simulink model "model"  (R2014a)
(part 4 of 5)

  _CN_227673096_110000_CN_53366641_110000/RConn3 -- T_53366641_220000;110000;6000_ПС_Канаш_220_110_6_кВ/RConn3 -- ВЛ_110_кВ_Канаш_Дружба_CN_53366641_110000_CN_207740804_110000/LConn3 -- ВЛ_110_кВ_Канаш_Дружба_CN_53366641_110000_CN_279846262_110000/LConn3 -- L_53366641/LConn3 -- bus24/LConn1 -- _CN_243154612_110000_CN_53366641_110000/LConn3 -- _CN_262366242_110000_CN_53366641_110000/LConn3 -- _CN_226054226_110000_CN_53366641_110000/LConn3 -- _CN_244847744_110000_CN_53366641_110000/LConn3
  _CN_198002186_110000_CN_197887411_110000/LConn1 -- T_198002186_110000;10000_ПС_110_10_кВ_Бройлерная/LConn1 -- _CN_198002186_110000_CN_311468947_110000/LConn1 -- _CN_198002186_110000_CN_234246987_110000/LConn1 -- _CN_198002186_110000_CN_281834842_110000/LConn1
  _CN_198002186_110000_CN_197887411_110000/LConn2 -- T_198002186_110000;10000_ПС_110_10_кВ_Бройлерная/LConn2 -- _CN_198002186_110000_CN_311468947_110000/LConn2 -- _CN_198002186_110000_CN_234246987_110000/LConn2 -- _CN_198002186_110000_CN_281834842_110000/LConn2
  _CN_198002186_110000_CN_197887411_110000/LConn3 -- T_198002186_110000;10000_ПС_110_10_кВ_Бройлерная/LConn3 -- _CN_198002186_110000_CN_311468947_110000/LConn3 -- _CN_198002186_110000_CN_234246987_110000/LConn3 -- _CN_198002186_110000_CN_281834842_110000/LConn3 -- bus25/LConn1
  _CN_198002186_110000_CN_197887411_110000/RConn1 -- T_197887411_110000;35000;10000_ПС_110_35_10_кВ_Атлашево/LConn1 -- _CN_313773134_110000_CN_197887411_110000/LConn1
  _CN_198002186_110000_CN_197887411_110000/RConn2 -- T_197887411_110000;35000;10000_ПС_110_35_10_кВ_Атлашево/LConn2 -- _CN_313773134_110000_CN_197887411_110000/LConn2
  _CN_198002186_110000_CN_197887411_110000/RConn3 -- T_197887411_110000;35000;10000_ПС_110_35_10_кВ_Атлашево/LConn3 -- _CN_313773134_110000_CN_197887411_110000/LConn3 -- bus26/LConn1
  _CN_198002186_110000_CN_311468947_110000/RConn1 -- T_311468947__ОРУ_ТЭЦ_3/LConn1 -- _CN_313773131_110000_CN_311468947_110000/LConn1 -- _CN_313773134_110000_CN_311468947_110000/LConn1
  _CN_198002186_110000_CN_311468947_110000/RConn2 -- T_311468947__ОРУ_ТЭЦ_3/LConn2 -- _CN_313773131_110000_CN_311468947_110000/LConn2 -- _CN_313773134_110000_CN_311468947_110000/LConn2
  _CN_198002186_110000_CN_311468947_110000/RConn3 -- T_311468947__ОРУ_ТЭЦ_3/LConn3 -- _CN_313773131_110000_CN_311468947_110000/LConn3 -- bus27/LConn1 -- _CN_313773134_110000_CN_311468947_110000/LConn3
  T_234246987_110000;10000_ПС_110_10_кВ_Луч/LConn1 -- _CN_198002186_110000_CN_234246987_110000/RConn1
  T_234246987_110000;10000_ПС_110_10_кВ_Луч/LConn2 -- _CN_198002186_110000_CN_234246987_110000/RConn2
  _CN_198002186_110000_CN_234246987_110000/RConn3 -- T_234246987_110000;10000_ПС_110_10_кВ_Луч/LConn3 -- bus28/LConn1
  _CN_198002186_110000_CN_281834842_110000/RConn1 -- T_281834842_110000;35000;10000_ПС_110_35_10_кВ_Катраси/LConn1 -- ВЛ_110_кВ_Южная_Катраси_CN_281834842_110000_CN_243075861_110000/LConn1 -- _CN_281834842_110000_CN_280247969_110000/RConn1 -- ВЛ_110_кВ_Катраси_Сундырь_с_отпайкой_Россия_CN_281834842_110000_CN_292328535_110000/LConn1 -- ВЛ_110_кВ_Катраси_Сундырь_с_отпайкой_Россия_CN_281834842_110000_CN_292068563_110000/LConn1 -- ВЛ_110_кВ_Катраси_Сундырь_с_отпайкой_Россия_CN_281834842_110000_CN_280247964_110000/LConn1 -- _CN_310752804_110000_CN_281834842_110000/LConn1 -- _CN_281834842_110000_CN_242972920_110000/LConn1 -- _CN_281834842_110000_CN_242973735_110000/LConn1
  _CN_198002186_110000_CN_281834842_110000/RConn2 -- T_281834842_110000;35000;10000_ПС_110_35_10_кВ_Катраси/LConn2 -- ВЛ_110_кВ_Южная_Катраси_CN_281834842_110000_CN_243075861_110000/LConn2 -- _CN_281834842_110000_CN_280247969_110000/RConn2 -- ВЛ_110_кВ_Катраси_Сундырь_с_отпайкой_Россия_CN_281834842_110000_CN_292328535_110000/LConn2 -- ВЛ_110_кВ_Катраси_Сундырь_с_отпайкой_Россия_CN_281834842_110000_CN_292068563_110000/LConn2 -- ВЛ_110_кВ_Катраси_Сундырь_с_отпайкой_Россия_CN_281834842_110000_CN_280247964_110000/LConn2 -- _CN_310752804_110000_CN_281834842_110000/LConn2 -- _CN_281834842_110000_CN_242972920_110000/LConn2 -- _CN_281834842_110000_CN_242973735_110000/LConn2
  _CN_198002186_110000_CN_281834842_110000/RConn3 -- T_281834842_110000;35000;10000_ПС_110_35_10_кВ_Катраси/LConn3 -- ВЛ_110_кВ_Южная_Катраси_CN_281834842_110000_CN_243075861_110000/LConn3 -- bus29/LConn1 -- _CN_281834842_110000_CN_280247969_110000/RConn3 -- ВЛ_110_кВ_Катраси_Сундырь_с_отпайкой_Россия_CN_281834842_110000_CN_292328535_110000/LConn3 -- ВЛ_110_кВ_Катраси_Сундырь_с_отпайкой_Россия_CN_281834842_110000_CN_292068563_110000/LConn3 -- ВЛ_110_кВ_Катраси_Сундырь_с_отпайкой_Россия_CN_281834842_110000_CN_280247964_110000/LConn3 -- _CN_310752804_110000_CN_281834842_110000/LConn3 -- _CN_281834842_110000_CN_242972920_110000/LConn3 -- _CN_281834842_110000_CN_242973735_110000/LConn3
  T_180390411__ПС_Бугульма/LConn1 -- ВЛ_Бугульма___Карабаш_II_110кВ_CN_180390411_110000_CN_238549570_110000/LConn1
  T_180390411__ПС_Бугульма/LConn2 -- ВЛ_Бугульма___Карабаш_II_110кВ_CN_180390411_110000_CN_238549570_110000/LConn2
  ВЛ_Бугульма___Карабаш_II_110кВ_CN_180390411_110000_CN_238549570_110000/LConn3 -- T_180390411__ПС_Бугульма/LConn3 -- bus30/LConn1
  T_238549570__ПС_Алкино/LConn1 -- ВЛ_Бугульма___Карабаш_II_110кВ_CN_180390411_110000_CN_238549570_110000/RConn1
  T_238549570__ПС_Алкино/LConn2 -- ВЛ_Бугульма___Карабаш_II_110кВ_CN_180390411_110000_CN_238549570_110000/RConn2
  ВЛ_Бугульма___Карабаш_II_110кВ_CN_180390411_110000_CN_238549570_110000/RConn3 -- T_238549570__ПС_Алкино/LConn3 -- bus31/LConn1
  T_82459148_110000_ОРУ_110_кВ/LConn1 -- _CN_82459148_110000_CN_273327356_110000/LConn1
  T_82459148_110000_ОРУ_110_кВ/LConn2 -- _CN_82459148_110000_CN_273327356_110000/LConn2
  _CN_82459148_110000_CN_273327356_110000/LConn3 -- T_82459148_110000_ОРУ_110_кВ/LConn3 -- bus32/LConn1
  _CN_82459148_110000_CN_273327356_110000/RConn1 -- G_273327356_Воткинская_ГЭС/RConn1 -- _CN_82458858_220000_CN_273327356_110000/LConn1 -- _CN_82459105_500000_CN_273327356_110000/LConn1
  _CN_82459148_110000_CN_273327356_110000/RConn2 -- G_273327356_Воткинская_ГЭС/RConn2 -- _CN_82458858_220000_CN_273327356_110000/LConn2 -- _CN_82459105_500000_CN_273327356_110000/LConn2
  _CN_82459148_110000_CN_273327356_110000/RConn3 -- G_273327356_Воткинская_ГЭС/RConn3 -- _CN_82458858_220000_CN_273327356_110000/LConn3 -- _CN_82459105_500000_CN_273327356_110000/LConn3 -- bus33/LConn1
  _CN_104554513_110000_CN_320965592_110000/LConn1 -- T_104554513__/LConn1 -- _CN_104554513_110000_CN_93482528_110000/LConn1 -- _CN_104554513_110000_CN_67498838_110000/RConn1
  _CN_104554513_110000_CN_320965592_110000/LConn2 -- T_104554513__/LConn2 -- _CN_104554513_110000_CN_93482528_110000/LConn2 -- _CN_104554513_110000_CN_67498838_110000/RConn2
  _CN_104554513_110000_CN_320965592_110000/LConn3 -- T_104554513__/LConn3 -- _CN_104554513_110000_CN_93482528_110000/LConn3 -- _CN_104554513_110000_CN_67498838_110000/RConn3 -- bus34/LConn1
  _CN_104554513_110000_CN_320965592_110000/RConn1 -- T_320965592__/LConn1 -- _CN_67498838_110000_CN_320965592_110000/RConn1
  _CN_104554513_110000_CN_320965592_110000/RConn2 -- T_320965592__/LConn2 -- _CN_67498838_110000_CN_320965592_110000/RConn2
  _CN_104554513_110000_CN_320965592_110000/RConn3 -- T_320965592__/LConn3 -- _CN_67498838_110000_CN_320965592_110000/RConn3 -- bus35/LConn1
  T_93482528__/LConn1 -- _CN_104554513_110000_CN_93482528_110000/RConn1
  T_93482528__/LConn2 -- _CN_104554513_110000_CN_93482528_110000/RConn2
  _CN_104554513_110000_CN_93482528_110000/RConn3 -- T_93482528__/LConn3 -- bus36/LConn1
  T_158349331__/LConn1 -- _CN_158349331_110000_CN_109525418_110000/LConn1
  T_158349331__/LConn2 -- _CN_158349331_110000_CN_109525418_110000/LConn2
  _CN_158349331_110000_CN_109525418_110000/LConn3 -- T_158349331__/LConn3 -- bus37/LConn1
  _CN_158349331_110000_CN_109525418_110000/RConn1 -- T_109525418_220000_Подстанция_220_кВ_Титан/LConn1 -- _CN_172819864_110000_CN_109525418_110000/LConn1 -- _CN_193928464_110000_CN_109525418_110000/LConn1 -- _CN_97060032_110000_CN_109525418_110000/LConn1 -- _CN_97060037_110000_CN_109525418_110000/LConn1
  _CN_158349331_110000_CN_109525418_110000/RConn2 -- T_109525418_220000_Подстанция_220_кВ_Титан/LConn2 -- _CN_172819864_110000_CN_109525418_110000/LConn2 -- _CN_193928464_110000_CN_109525418_110000/LConn2 -- _CN_97060032_110000_CN_109525418_110000/LConn2 -- _CN_97060037_110000_CN_109525418_110000/LConn2
  _CN_158349331_110000_CN_109525418_110000/RConn3 -- T_109525418_220000_Подстанция_220_кВ_Титан/LConn3 -- _CN_172819864_110000_CN_109525418_110000/LConn3 -- bus38/LConn1 -- _CN_193928464_110000_CN_109525418_110000/LConn3 -- _CN_97060032_110000_CN_109525418_110000/LConn3 -- _CN_97060037_110000_CN_109525418_110000/LConn3
  T_330052123_110000_ПС_110_6_кВ_Прудовая/LConn1 -- _CN_330052123_110000_CN_116695201_110000/LConn1
  T_330052123_110000_ПС_110_6_кВ_Прудовая/LConn2 -- _CN_330052123_110000_CN_116695201_110000/LConn2
  _CN_330052123_110000_CN_116695201_110000/LConn3 -- T_330052123_110000_ПС_110_6_кВ_Прудовая/LConn3 -- bus39/LConn1
  _CN_330052123_110000_CN_116695201_110000/RConn1 -- T_116695201_110000_ПС_110_35_6_Воткинск/LConn1 -- _CN_330006647_110000_CN_116695201_110000/LConn1 -- _CN_172508720_110000_CN_116695201_110000/LConn1
  _CN_330052123_110000_CN_116695201_110000/RConn2 -- T_116695201_110000_ПС_110_35_6_Воткинск/LConn2 -- _CN_330006647_110000_CN_116695201_110000/LConn2 -- _CN_172508720_110000_CN_116695201_110000/LConn2
  _CN_330052123_110000_CN_116695201_110000/RConn3 -- T_116695201_110000_ПС_110_35_6_Воткинск/LConn3 -- _CN_330006647_110000_CN_116695201_110000/LConn3 -- bus40/LConn1 -- _CN_172508720_110000_CN_116695201_110000/LConn3
  _CN_262366242_110000_CN_208425687_110000/LConn1 -- T_262366242_110000;35000;10000_ПС_110_35_10_кВ_Батырево/LConn1 -- _CN_262366242_110000_CN_53366641_110000/RConn1 -- _CN_262366242_110000_CN_243068515_110000/LConn1 -- _CN_262366242_110000_CN_279919300_110000/RConn1 -- _CN_262366242_110000_CN_262366241_110000/LConn1
  _CN_262366242_110000_CN_208425687_110000/LConn2 -- T_262366242_110000;35000;10000_ПС_110_35_10_кВ_Батырево/LConn2 -- _CN_262366242_110000_CN_53366641_110000/RConn2 -- _CN_262366242_110000_CN_243068515_110000/LConn2 -- _CN_262366242_110000_CN_279919300_110000/RConn2 -- _CN_262366242_110000_CN_262366241_110000/LConn2
  _CN_262366242_110000_CN_208425687_110000/LConn3 -- T_262366242_110000;35000;10000_ПС_110_35_10_кВ_Батырево/LConn3 -- _CN_262366242_110000_CN_53366641_110000/RConn3 -- _CN_262366242_110000_CN_243068515_110000/LConn3 -- _CN_262366242_110000_CN_279919300_110000/RConn3 -- _CN_262366242_110000_CN_262366241_110000/LConn3 -- bus41/LConn1
  T_208425687_110000;35000;10000_ПС_110_35_10_кВ_Комсомольская/LConn1 -- _CN_262366242_110000_CN_208425687_110000/RConn1
  T_208425687_110000;35000;10000_ПС_110_35_10_кВ_Комсомольская/LConn2 -- _CN_262366242_110000_CN_208425687_110000/RConn2
  _CN_262366242_110000_CN_208425687_110000/RConn3 -- T_208425687_110000;35000;10000_ПС_110_35_10_кВ_Комсомольская/LConn3 -- bus42/LConn1
  T_243068515_110000;10000_ПС_110_10_кВ_Маяк/LConn1 -- _CN_262366242_110000_CN_243068515_110000/RConn1
  T_243068515_110000;10000_ПС_110_10_кВ_Маяк/LConn2 -- _CN_262366242_110000_CN_243068515_110000/RConn2
  _CN_262366242_110000_CN_243068515_110000/RConn3 -- T_243068515_110000;10000_ПС_110_10_кВ_Маяк/LConn3 -- bus43/LConn1
  _CN_262366242_110000_CN_262366241_110000/RConn1 -- T_262366241_110000;10000_ПС_110_10_кВ_Сугуты/LConn1 -- _CN_194431022_110000_CN_262366241_110000/LConn1
  _CN_262366242_110000_CN_262366241_110000/RConn2 -- T_262366241_110000;10000_ПС_110_10_кВ_Сугуты/LConn2 -- _CN_194431022_110000_CN_262366241_110000/LConn2
  _CN_262366242_110000_CN_262366241_110000/RConn3 -- T_262366241_110000;10000_ПС_110_10_кВ_Сугуты/LConn3 -- _CN_194431022_110000_CN_262366241_110000/LConn3 -- bus44/LConn1
  _CN_310752804_110000_CN_281834842_110000/RConn1 -- T_310752804_110000;35000;10000_ПС_«Чапаевская»_110_35_10_кВ/LConn1 -- _CN_310752804_110000_CN_243075861_110000/LConn1
  _CN_310752804_110000_CN_281834842_110000/RConn2 -- T_310752804_110000;35000;10000_ПС_«Чапаевская»_110_35_10_кВ/LConn2 -- _CN_310752804_110000_CN_243075861_110000/LConn2
  _CN_310752804_110000_CN_281834842_110000/RConn3 -- T_310752804_110000;35000;10000_ПС_«Чапаевская»_110_35_10_кВ/LConn3 -- _CN_310752804_110000_CN_243075861_110000/LConn3 -- bus45/LConn1
  _CN_310752804_110000_CN_243075861_110000/RConn1 -- T_243075861_110000;6000_ПС_110_6_кВ_Южная/LConn1 -- ВЛ_110_кВ_Южная_Катраси_CN_281834842_110000_CN_243075861_110000/RConn1
  _CN_310752804_110000_CN_243075861_110000/RConn2 -- T_243075861_110000;6000_ПС_110_6_кВ_Южная/LConn2 -- ВЛ_110_кВ_Южная_Катраси_CN_281834842_110000_CN_243075861_110000/RConn2
  _CN_310752804_110000_CN_243075861_110000/RConn3 -- T_243075861_110000;6000_ПС_110_6_кВ_Южная/LConn3 -- ВЛ_110_кВ_Южная_Катраси_CN_281834842_110000_CN_243075861_110000/RConn3 -- bus46/LConn1
  _CN_97124903_110000_CN_145399632_110000/LConn1 -- T_97124903__/LConn1 -- _CN_97124903_110000_CN_97124768_110000/LConn1
  _CN_97124903_110000_CN_145399632_110000/LConn2 -- T_97124903__/LConn2 -- _CN_97124903_110000_CN_97124768_110000/LConn2
  _CN_97124903_110000_CN_145399632_110000/LConn3 -- T_97124903__/LConn3 -- _CN_97124903_110000_CN_97124768_110000/LConn3 -- bus47/LConn1
  T_145399632__/LConn1 -- _CN_97124903_110000_CN_145399632_110000/RConn1
  T_145399632__/LConn2 -- _CN_97124903_110000_CN_145399632_110000/RConn2
  _CN_97124903_110000_CN_145399632_110000/RConn3 -- T_145399632__/LConn3 -- bus48/LConn1
  T_97124768__/LConn1 -- _CN_97124903_110000_CN_97124768_110000/RConn1
  T_97124768__/LConn2 -- _CN_97124903_110000_CN_97124768_110000/RConn2
  _CN_97124903_110000_CN_97124768_110000/RConn3 -- T_97124768__/LConn3 -- bus49/LConn1
  _CN_279978588_110000_CN_279978582_110000/LConn1 -- T_279978588_110000;10000_ПС_110_10_кВ_Алгаши/LConn1 -- _CN_279978588_110000_CN_279978583_110000/LConn1 -- _CN_279978588_110000_CN_207204995_110000/LConn1
  _CN_279978588_110000_CN_279978582_110000/LConn2 -- T_279978588_110000;10000_ПС_110_10_кВ_Алгаши/LConn2 -- _CN_279978588_110000_CN_279978583_110000/LConn2 -- _CN_279978588_110000_CN_207204995_110000/LConn2
  _CN_279978588_110000_CN_279978582_110000/LConn3 -- T_279978588_110000;10000_ПС_110_10_кВ_Алгаши/LConn3 -- _CN_279978588_110000_CN_279978583_110000/LConn3 -- _CN_279978588_110000_CN_207204995_110000/LConn3 -- bus50/LConn1
  _CN_279978588_110000_CN_279978582_110000/RConn1 -- T_279978582_110000;35000;10000_ПС_110_35_10_кВ_Порецкая/LConn1 -- _CN_279978581_110000_CN_279978582_110000/LConn1
  _CN_279978588_110000_CN_279978582_110000/RConn2 -- T_279978582_110000;35000;10000_ПС_110_35_10_кВ_Порецкая/LConn2 -- _CN_279978581_110000_CN_279978582_110000/LConn2
  _CN_279978588_110000_CN_279978582_110000/RConn3 -- T_279978582_110000;35000;10000_ПС_110_35_10_кВ_Порецкая/LConn3 -- _CN_279978581_110000_CN_279978582_110000/LConn3 -- bus51/LConn1
  T_279978583_110000;10000_ПС_110_10_кВ_Кожевенная/LConn1 -- _CN_279978588_110000_CN_279978583_110000/RConn1
  T_279978583_110000;10000_ПС_110_10_кВ_Кожевенная/LConn2 -- _CN_279978588_110000_CN_279978583_110000/RConn2
  _CN_279978588_110000_CN_279978583_110000/RConn3 -- T_279978583_110000;10000_ПС_110_10_кВ_Кожевенная/LConn3 -- bus52/LConn1
  _CN_279978588_110000_CN_207204995_110000/RConn1 -- T_207204995_220000;110000;6000_ПС_Венец_220_110_6_кВ/RConn1 -- _CN_244847744_110000_CN_207204995_110000/LConn1 -- _CN_207204995_110000_CN_207206840_110000/LConn1 -- L_207204995/LConn1
  _CN_279978588_110000_CN_207204995_110000/RConn2 -- T_207204995_220000;110000;6000_ПС_Венец_220_110_6_кВ/RConn2 -- _CN_244847744_110000_CN_207204995_110000/LConn2 -- _CN_207204995_110000_CN_207206840_110000/LConn2 -- L_207204995/LConn2
  _CN_279978588_110000_CN_207204995_110000/RConn3 -- T_207204995_220000;110000;6000_ПС_Венец_220_110_6_кВ/RConn3 -- _CN_244847744_110000_CN_207204995_110000/LConn3 -- _CN_207204995_110000_CN_207206840_110000/LConn3 -- L_207204995/LConn3 -- bus53/LConn1
  _CN_250911823_110000_CN_351596015_110000/LConn1 -- T_250911823__ПС_Б_Матаки/LConn1 -- _CN_250911823_110000_CN_183273018_110000/LConn1
  _CN_250911823_110000_CN_351596015_110000/LConn2 -- T_250911823__ПС_Б_Матаки/LConn2 -- _CN_250911823_110000_CN_183273018_110000/LConn2
  _CN_250911823_110000_CN_351596015_110000/LConn3 -- T_250911823__ПС_Б_Матаки/LConn3 -- _CN_250911823_110000_CN_183273018_110000/LConn3 -- bus54/LConn1
  T_351596015__ПС_Ромодан/LConn1 -- _CN_250911823_110000_CN_351596015_110000/RConn1
  T_351596015__ПС_Ромодан/LConn2 -- _CN_250911823_110000_CN_351596015_110000/RConn2
  _CN_250911823_110000_CN_351596015_110000/RConn3 -- T_351596015__ПС_Ромодан/LConn3 -- bus55/LConn1
  T_183273018__ПС_Салманы/LConn1 -- _CN_250911823_110000_CN_183273018_110000/RConn1
  T_183273018__ПС_Салманы/LConn2 -- _CN_250911823_110000_CN_183273018_110000/RConn2
  _CN_250911823_110000_CN_183273018_110000/RConn3 -- T_183273018__ПС_Салманы/LConn3 -- bus56/LConn1
  _CN_194431022_110000_CN_262366241_110000/RConn1 -- T_194431022_110000;35000;10000_ПС_110_35_10_кВ_Яльчики/LConn1 -- _CN_194431022_110000_CN_279778884_110000/LConn1
  _CN_194431022_110000_CN_262366241_110000/RConn2 -- T_194431022_110000;35000;10000_ПС_110_35_10_кВ_Яльчики/LConn2 -- _CN_194431022_110000_CN_279778884_110000/LConn2
  _CN_194431022_110000_CN_262366241_110000/RConn3 -- T_194431022_110000;35000;10000_ПС_110_35_10_кВ_Яльчики/LConn3 -- _CN_194431022_110000_CN_279778884_110000/LConn3 -- bus57/LConn1
  T_279778884_110000;10000_ПС_110_10_кВ_Слава/LConn1 -- _CN_194431022_110000_CN_279778884_110000/RConn1
  T_279778884_110000;10000_ПС_110_10_кВ_Слава/LConn2 -- _CN_194431022_110000_CN_279778884_110000/RConn2
  _CN_194431022_110000_CN_279778884_110000/RConn3 -- T_279778884_110000;10000_ПС_110_10_кВ_Слава/LConn3 -- bus58/LConn1
  T_172508720_110000_ПС_110_10_Успенка/LConn1 -- _CN_172508720_110000_CN_116695201_110000/RConn1
  T_172508720_110000_ПС_110_10_Успенка/LConn2 -- _CN_172508720_110000_CN_116695201_110000/RConn2
  _CN_172508720_110000_CN_116695201_110000/RConn3 -- T_172508720_110000_ПС_110_10_Успенка/LConn3 -- bus59/LConn1
  _CN_157080628_110000_CN_192432407_110000/LConn1 -- T_157080628__/LConn1 -- _CN_157080628_110000_CN_192432406_110000/LConn1 -- _CN_157080628_110000_CN_192426717_110000/LConn1
  _CN_157080628_110000_CN_192432407_110000/LConn2 -- T_157080628__/LConn2 -- _CN_157080628_110000_CN_192432406_110000/LConn2 -- _CN_157080628_110000_CN_192426717_110000/LConn2
  _CN_157080628_110000_CN_192432407_110000/LConn3 -- T_157080628__/LConn3 -- _CN_157080628_110000_CN_192432406_110000/LConn3 -- _CN_157080628_110000_CN_192426717_110000/LConn3 -- bus60/LConn1
  T_192432407__/LConn1 -- _CN_157080628_110000_CN_192432407_110000/RConn1
  T_192432407__/LConn2 -- _CN_157080628_110000_CN_192432407_110000/RConn2
  _CN_157080628_110000_CN_192432407_110000/RConn3 -- T_192432407__/LConn3 -- bus61/LConn1
  T_192432406__/LConn1 -- _CN_157080628_110000_CN_192432406_110000/RConn1
  T_192432406__/LConn2 -- _CN_157080628_110000_CN_192432406_110000/RConn2
  _CN_157080628_110000_CN_192432406_110000/RConn3 -- T_192432406__/LConn3 -- bus62/LConn1
  T_192426717_110000_ПС_Люзень/LConn1 -- _CN_157080628_110000_CN_192426717_110000/RConn1
  T_192426717_110000_ПС_Люзень/LConn2 -- _CN_157080628_110000_CN_192426717_110000/RConn2
  _CN_157080628_110000_CN_192426717_110000/RConn3 -- T_192426717_110000_ПС_Люзень/LConn3 -- bus63/LConn1
  T_236703070__ПС_Дубъязы/LConn1 -- ВЛ_Дубъязы___Алат_110кВ_CN_236703070_110000_CN_180786877_110000/LConn1
  T_236703070__ПС_Дубъязы/LConn2 -- ВЛ_Дубъязы___Алат_110кВ_CN_236703070_110000_CN_180786877_110000/LConn2
  ВЛ_Дубъязы___Алат_110кВ_CN_236703070_110000_CN_180786877_110000/LConn3 -- T_236703070__ПС_Дубъязы/LConn3 -- bus64/LConn1
  T_180786877__ПС_Алат/LConn1 -- ВЛ_Дубъязы___Алат_110кВ_CN_236703070_110000_CN_180786877_110000/RConn1
  T_180786877__ПС_Алат/LConn2 -- ВЛ_Дубъязы___Алат_110кВ_CN_236703070_110000_CN_180786877_110000/RConn2
  ВЛ_Дубъязы___Алат_110кВ_CN_236703070_110000_CN_180786877_110000/RConn3 -- T_180786877__ПС_Алат/LConn3 -- bus65/LConn1
  T_291372086_110000_пс_Села_110_10кВ/LConn1 -- _CN_291372086_110000_CN_291372085_110000/LConn1
  T_291372086_110000_пс_Села_110_10кВ/LConn2 -- _CN_291372086_110000_CN_291372085_110000/LConn2
  _CN_291372086_110000_CN_291372085_110000/LConn3 -- T_291372086_110000_пс_Села_110_10кВ/LConn3 -- bus66/LConn1
  T_291372085_110000_пс_Кутамыш/LConn1 -- _CN_291372086_110000_CN_291372085_110000/RConn1
  T_291372085_110000_пс_Кутамыш/LConn2 -- _CN_291372086_110000_CN_291372085_110000/RConn2
  _CN_291372086_110000_CN_291372085_110000/RConn3 -- T_291372085_110000_пс_Кутамыш/LConn3 -- bus67/LConn1
  _CN_277905350_110000_CN_277905349_110000/LConn1 -- T_277905350_220000;110000_Сергач/RConn1 -- L_277905350/LConn1
  _CN_277905350_110000_CN_277905349_110000/LConn2 -- T_277905350_220000;110000_Сергач/RConn2 -- L_277905350/LConn2
  _CN_277905350_110000_CN_277905349_110000/LConn3 -- T_277905350_220000;110000_Сергач/RConn3 -- L_277905350/LConn3 -- bus68/LConn1
  T_277905349_110000;10000_Андреевка/LConn1 -- _CN_277905350_110000_CN_277905349_110000/RConn1
  T_277905349_110000;10000_Андреевка/LConn2 -- _CN_277905350_110000_CN_277905349_110000/RConn2
  _CN_277905350_110000_CN_277905349_110000/RConn3 -- T_277905349_110000;10000_Андреевка/LConn3 -- bus69/LConn1
  _CN_281834842_110000_CN_242972920_110000/RConn1 -- T_242972920_110000;10000_ПС_110_10_кВ_Заволжская/LConn1 -- _CN_279258960_110000_CN_242972920_110000/LConn1
  _CN_281834842_110000_CN_242972920_110000/RConn2 -- T_242972920_110000;10000_ПС_110_10_кВ_Заволжская/LConn2 -- _CN_279258960_110000_CN_242972920_110000/LConn2
  _CN_281834842_110000_CN_242972920_110000/RConn3 -- T_242972920_110000;10000_ПС_110_10_кВ_Заволжская/LConn3 -- _CN_279258960_110000_CN_242972920_110000/LConn3 -- bus70/LConn1
  T_242973735_110000;10000_ПС_110_10_кВ_Яндоба/LConn1 -- _CN_281834842_110000_CN_242973735_110000/RConn1
  T_242973735_110000;10000_ПС_110_10_кВ_Яндоба/LConn2 -- _CN_281834842_110000_CN_242973735_110000/RConn2
  _CN_281834842_110000_CN_242973735_110000/RConn3 -- T_242973735_110000;10000_ПС_110_10_кВ_Яндоба/LConn3 -- bus71/LConn1
  T_292328535_110000;10000_ПС_110_10_кВ_Виловатово/LConn1 -- ВЛ_110_кВ_Катраси_Сундырь_с_отпайкой_Россия_CN_281834842_110000_CN_292328535_110000/RConn1
  T_292328535_110000;10000_ПС_110_10_кВ_Виловатово/LConn2 -- ВЛ_110_кВ_Катраси_Сундырь_с_отпайкой_Россия_CN_281834842_110000_CN_292328535_110000/RConn2
  ВЛ_110_кВ_Катраси_Сундырь_с_отпайкой_Россия_CN_281834842_110000_CN_292328535_110000/RConn3 -- T_292328535_110000;10000_ПС_110_10_кВ_Виловатово/LConn3 -- bus72/LConn1
  T_292068563_110000;35000;10000_ПС_110_35_10_кВ_Еласы/LConn1 -- ВЛ_110_кВ_Катраси_Сундырь_с_отпайкой_Россия_CN_281834842_110000_CN_292068563_110000/RConn1
  T_292068563_110000;35000;10000_ПС_110_35_10_кВ_Еласы/LConn2 -- ВЛ_110_кВ_Катраси_Сундырь_с_отпайкой_Россия_CN_281834842_110000_CN_292068563_110000/RConn2
  ВЛ_110_кВ_Катраси_Сундырь_с_отпайкой_Россия_CN_281834842_110000_CN_292068563_110000/RConn3 -- T_292068563_110000;35000;10000_ПС_110_35_10_кВ_Еласы/LConn3 -- bus73/LConn1
  T_280247964_110000;10000_ПС_110_10_кВ_Сундырь/LConn1 -- ВЛ_110_кВ_Катраси_Сундырь_с_отпайкой_Россия_CN_281834842_110000_CN_280247964_110000/RConn1
  T_280247964_110000;10000_ПС_110_10_кВ_Сундырь/LConn2 -- ВЛ_110_кВ_Катраси_Сундырь_с_отпайкой_Россия_CN_281834842_110000_CN_280247964_110000/RConn2
  ВЛ_110_кВ_Катраси_Сундырь_с_отпайкой_Россия_CN_281834842_110000_CN_280247964_110000/RConn3 -- T_280247964_110000;10000_ПС_110_10_кВ_Сундырь/LConn3 -- bus74/LConn1
  T_226055229_110000;10000_ПС_110_10_кВ_Козловка/LConn1 -- ВЛ_Тюрлема___Козловка_110кВ_CN_226055229_110000_CN_121218185_110000/LConn1
  T_226055229_110000;10000_ПС_110_10_кВ_Козловка/LConn2 -- ВЛ_Тюрлема___Козловка_110кВ_CN_226055229_110000_CN_121218185_110000/LConn2
  ВЛ_Тюрлема___Козловка_110кВ_CN_226055229_110000_CN_121218185_110000/LConn3 -- T_226055229_110000;10000_ПС_110_10_кВ_Козловка/LConn3 -- bus75/LConn1
  ВЛ_Тюрлема___Козловка_110кВ_CN_226055229_110000_CN_121218185_110000/RConn1 -- T_121218185_220000;110000;10000_ПС_220_110_10_кВ_Тюрлема/RConn1 -- _CN_121218185_110000_CN_226055643_110000/LConn1 -- L_121218185/LConn1 -- ВЛ_Свияжск___Тюрлема_110кВ_CN_121218185_110000_CN_191841753_110000/LConn1 -- ВЛ_Нурлаты___Федоровская_110_кВ_CN_120823877_110000_CN_121218185_110000/LConn1 -- _CN_226054226_110000_CN_121218185_110000/LConn1
  ВЛ_Тюрлема___Козловка_110кВ_CN_226055229_110000_CN_121218185_110000/RConn2 -- T_121218185_220000;110000;10000_ПС_220_110_10_кВ_Тюрлема/RConn2 -- _CN_121218185_110000_CN_226055643_110000/LConn2 -- L_121218185/LConn2 -- ВЛ_Свияжск___Тюрлема_110кВ_CN_121218185_110000_CN_191841753_110000/LConn2 -- ВЛ_Нурлаты___Федоровская_110_кВ_CN_120823877_110000_CN_121218185_110000/LConn2 -- _CN_226054226_110000_CN_121218185_110000/LConn2
  ВЛ_Тюрлема___Козловка_110кВ_CN_226055229_110000_CN_121218185_110000/RConn3 -- T_121218185_220000;110000;10000_ПС_220_110_10_кВ_Тюрлема/RConn3 -- _CN_121218185_110000_CN_226055643_110000/LConn3 -- L_121218185/LConn3 -- bus76/LConn1 -- ВЛ_Свияжск___Тюрлема_110кВ_CN_121218185_110000_CN_191841753_110000/LConn3 -- ВЛ_Нурлаты___Федоровская_110_кВ_CN_120823877_110000_CN_121218185_110000/LConn3 -- _CN_226054226_110000_CN_121218185_110000/LConn3
  _CN_115651649_110000_CN_281879368_110000/LConn1 -- T_115651649_110000;10000_ПС_110_10_кВ_Вурманкасы/LConn1 -- _CN_115651649_110000_CN_281834847_110000/LConn1
  _CN_115651649_110000_CN_281879368_110000/LConn2 -- T_115651649_110000;10000_ПС_110_10_кВ_Вурманкасы/LConn2 -- _CN_115651649_110000_CN_281834847_110000/LConn2
  _CN_115651649_110000_CN_281879368_110000/LConn3 -- T_115651649_110000;10000_ПС_110_10_кВ_Вурманкасы/LConn3 -- _CN_115651649_110000_CN_281834847_110000/LConn3 -- bus77/LConn1
  T_281879368_110000;10000_ПС_110_10_кВ_Радуга/LConn1 -- _CN_115651649_110000_CN_281879368_110000/RConn1
  T_281879368_110000;10000_ПС_110_10_кВ_Радуга/LConn2 -- _CN_115651649_110000_CN_281879368_110000/RConn2
  _CN_115651649_110000_CN_281879368_110000/RConn3 -- T_281879368_110000;10000_ПС_110_10_кВ_Радуга/LConn3 -- bus78/LConn1
  T_281834847_110000;35000;10000_ПС_110_35_10_кВ_Кугеси/LConn1 -- _CN_115651649_110000_CN_281834847_110000/RConn1
  T_281834847_110000;35000;10000_ПС_110_35_10_кВ_Кугеси/LConn2 -- _CN_115651649_110000_CN_281834847_110000/RConn2
  _CN_115651649_110000_CN_281834847_110000/RConn3 -- T_281834847_110000;35000;10000_ПС_110_35_10_кВ_Кугеси/LConn3 -- bus79/LConn1
  ВЛ_Нурлаты___Федоровская_110_кВ_CN_120823877_110000_CN_229841888_110000/LConn1 -- T_120823877__ПС_Федоровская/LConn1 -- ВЛ_Нурлаты___Федоровская_110_кВ_CN_120823877_110000_CN_121218185_110000/RConn1 -- ВЛ_Нурлаты___Федоровская_110_кВ_CN_120823877_110000_CN_171977680_110000/LConn1 -- ВЛ_Нурлаты___Федоровская_110_кВ_CN_120823877_110000_CN_176838936_110000/LConn1
  ВЛ_Нурлаты___Федоровская_110_кВ_CN_120823877_110000_CN_229841888_110000/LConn2 -- T_120823877__ПС_Федоровская/LConn2 -- ВЛ_Нурлаты___Федоровская_110_кВ_CN_120823877_110000_CN_121218185_110000/RConn2 -- ВЛ_Нурлаты___Федоровская_110_кВ_CN_120823877_110000_CN_171977680_110000/LConn2 -- ВЛ_Нурлаты___Федоровская_110_кВ_CN_120823877_110000_CN_176838936_110000/LConn2
  ВЛ_Нурлаты___Федоровская_110_кВ_CN_120823877_110000_CN_229841888_110000/LConn3 -- T_120823877__ПС_Федоровская/LConn3 -- ВЛ_Нурлаты___Федоровская_110_кВ_CN_120823877_110000_CN_121218185_110000/RConn3 -- ВЛ_Нурлаты___Федоровская_110_кВ_CN_120823877_110000_CN_171977680_110000/LConn3 -- ВЛ_Нурлаты___Федоровская_110_кВ_CN_120823877_110000_CN_176838936_110000/LConn3 -- bus80/LConn1
  T_229841888__ПС_Нурлаты/LConn1 -- ВЛ_Нурлаты___Федоровская_110_кВ_CN_120823877_110000_CN_229841888_110000/RConn1
  T_229841888__ПС_Нурлаты/LConn2 -- ВЛ_Нурлаты___Федоровская_110_кВ_CN_120823877_110000_CN_229841888_110000/RConn2
  ВЛ_Нурлаты___Федоровская_110_кВ_CN_120823877_110000_CN_229841888_110000/RConn3 -- T_229841888__ПС_Нурлаты/LConn3 -- bus81/LConn1
  ВЛ_Нурлаты___Федоровская_110_кВ_CN_120823877_110000_CN_171977680_110000/RConn1 -- T_171977680__ПС_Апастово/LConn1 -- _CN_113994637_110000_CN_171977680_110000/LConn1
  ВЛ_Нурлаты___Федоровская_110_кВ_CN_120823877_110000_CN_171977680_110000/RConn2 -- T_171977680__ПС_Апастово/LConn2 -- _CN_113994637_110000_CN_171977680_110000/LConn2
  ВЛ_Нурлаты___Федоровская_110_кВ_CN_120823877_110000_CN_171977680_110000/RConn3 -- T_171977680__ПС_Апастово/LConn3 -- _CN_113994637_110000_CN_171977680_110000/LConn3 -- bus82/LConn1
  T_176838936__ПС_Каратун/LConn1 -- ВЛ_Нурлаты___Федоровская_110_кВ_CN_120823877_110000_CN_176838936_110000/RConn1
  T_176838936__ПС_Каратун/LConn2 -- ВЛ_Нурлаты___Федоровская_110_кВ_CN_120823877_110000_CN_176838936_110000/RConn2
  ВЛ_Нурлаты___Федоровская_110_кВ_CN_120823877_110000_CN_176838936_110000/RConn3 -- T_176838936__ПС_Каратун/LConn3 -- bus83/LConn1
  T_94242892__Подстанция_№3/LConn1 -- _CN_94242892_110000_CN_97145033_110000/LConn1
  T_94242892__Подстанция_№3/LConn2 -- _CN_94242892_110000_CN_97145033_110000/LConn2
  _CN_94242892_110000_CN_97145033_110000/LConn3 -- T_94242892__Подстанция_№3/LConn3 -- bus84/LConn1
  _CN_94242892_110000_CN_97145033_110000/RConn1 -- T_97145033_220000;110000;10000_ПС_220_кВ_Орская/RConn1 -- L_97145033/LConn1
  _CN_94242892_110000_CN_97145033_110000/RConn2 -- T_97145033_220000;110000;10000_ПС_220_кВ_Орская/RConn2 -- L_97145033/LConn2
  _CN_94242892_110000_CN_97145033_110000/RConn3 -- T_97145033_220000;110000;10000_ПС_220_кВ_Орская/RConn3 -- L_97145033/LConn3 -- bus85/LConn1
  110_кВ_CN_138632781_110000_CN_138722426_110000/LConn1 -- "T_138632781_220000;110000;10000_ПС_220_110_10_кВ_\"Сасово\""/LConn1 -- 110_кВ_CN_138632781_110000_CN_140944227_110000/LConn1 -- 110_кВ_CN_138632781_110000_CN_140940409_110000/LConn1 -- 110_кВ_CN_138632781_110000_CN_181334375_110000/LConn1
  110_кВ_CN_138632781_110000_CN_138722426_110000/LConn2 -- "T_138632781_220000;110000;10000_ПС_220_110_10_кВ_\"Сасово\""/LConn2 -- 110_кВ_CN_138632781_110000_CN_140944227_110000/LConn2 -- 110_кВ_CN_138632781_110000_CN_140940409_110000/LConn2 -- 110_кВ_CN_138632781_110000_CN_181334375_110000/LConn2
  110_кВ_CN_138632781_110000_CN_138722426_110000/LConn3 -- "T_138632781_220000;110000;10000_ПС_220_110_10_кВ_\"Сасово\""/LConn3 -- 110_кВ_CN_138632781_110000_CN_140944227_110000/LConn3 -- 110_кВ_CN_138632781_110000_CN_140940409_110000/LConn3 -- 110_кВ_CN_138632781_110000_CN_181334375_110000/LConn3 -- bus86/LConn1
  "T_138722426__ПС_110_10кВ_\"Вад\""/LConn1 -- 110_кВ_CN_138632781_110000_CN_138722426_110000/RConn1
  "T_138722426__ПС_110_10кВ_\"Вад\""/LConn2 -- 110_кВ_CN_138632781_110000_CN_138722426_110000/RConn2
  110_кВ_CN_138632781_110000_CN_138722426_110000/RConn3 -- "T_138722426__ПС_110_10кВ_\"Вад\""/LConn3 -- bus87/LConn1
  T_140944227__/LConn1 -- 110_кВ_CN_138632781_110000_CN_140944227_110000/RConn1
  T_140944227__/LConn2 -- 110_кВ_CN_138632781_110000_CN_140944227_110000/RConn2
  110_кВ_CN_138632781_110000_CN_140944227_110000/RConn3 -- T_140944227__/LConn3 -- bus88/LConn1
  "T_140940409_110000;10000_ПС_110_10_кВ_\"Свобода\""/LConn1 -- 110_кВ_CN_138632781_110000_CN_140940409_110000/RConn1
  "T_140940409_110000;10000_ПС_110_10_кВ_\"Свобода\""/LConn2 -- 110_кВ_CN_138632781_110000_CN_140940409_110000/RConn2
  110_кВ_CN_138632781_110000_CN_140940409_110000/RConn3 -- "T_140940409_110000;10000_ПС_110_10_кВ_\"Свобода\""/LConn3 -- bus89/LConn1
  "T_181334375__ПС_110_10кВ_\"Кустаревка\""/LConn1 -- 110_кВ_CN_138632781_110000_CN_181334375_110000/RConn1
  "T_181334375__ПС_110_10кВ_\"Кустаревка\""/LConn2 -- 110_кВ_CN_138632781_110000_CN_181334375_110000/RConn2
  110_кВ_CN_138632781_110000_CN_181334375_110000/RConn3 -- "T_181334375__ПС_110_10кВ_\"Кустаревка\""/LConn3 -- bus90/LConn1
  _CN_313773134_110000_CN_197887411_110000/RConn1 -- T_313773134_110000;35000;6000_ПС_110_35_6_кВ_Порт/LConn1 -- _CN_313773134_110000_CN_311468947_110000/RConn1 -- _CN_313773134_110000_CN_313773131_110000/LConn1
  _CN_313773134_110000_CN_197887411_110000/RConn2 -- T_313773134_110000;35000;6000_ПС_110_35_6_кВ_Порт/LConn2 -- _CN_313773134_110000_CN_311468947_110000/RConn2 -- _CN_313773134_110000_CN_313773131_110000/LConn2
  _CN_313773134_110000_CN_197887411_110000/RConn3 -- T_313773134_110000;35000;6000_ПС_110_35_6_кВ_Порт/LConn3 -- _CN_313773134_110000_CN_311468947_110000/RConn3 -- _CN_313773134_110000_CN_313773131_110000/LConn3 -- bus91/LConn1
  _CN_313773134_110000_CN_313773131_110000/RConn1 -- T_313773131__/LConn1 -- _CN_313773131_110000_CN_281879365_110000/LConn1 -- _CN_313773131_110000_CN_311468947_110000/RConn1 -- _CN_313773131_110000_CN_58880346_110000/LConn1
  _CN_313773134_110000_CN_313773131_110000/RConn2 -- T_313773131__/LConn2 -- _CN_313773131_110000_CN_281879365_110000/LConn2 -- _CN_313773131_110000_CN_311468947_110000/RConn2 -- _CN_313773131_110000_CN_58880346_110000/LConn2
  _CN_313773134_110000_CN_313773131_110000/RConn3 -- T_313773131__/LConn3 -- _CN_313773131_110000_CN_281879365_110000/LConn3 -- bus92/LConn1 -- _CN_313773131_110000_CN_311468947_110000/RConn3 -- _CN_313773131_110000_CN_58880346_110000/LConn3
  _CN_226054226_110000_CN_226052064_110000/LConn1 -- T_226054226_110000;10000_ПС_110_10_кВ_Кибечи/LConn1 -- _CN_226054226_110000_CN_243069892_110000/LConn1 -- _CN_226054226_110000_CN_121218185_110000/RConn1 -- _CN_226054226_110000_CN_53366641_110000/RConn1
  _CN_226054226_110000_CN_226052064_110000/LConn2 -- T_226054226_110000;10000_ПС_110_10_кВ_Кибечи/LConn2 -- _CN_226054226_110000_CN_243069892_110000/LConn2 -- _CN_226054226_110000_CN_121218185_110000/RConn2 -- _CN_226054226_110000_CN_53366641_110000/RConn2
  _CN_226054226_110000_CN_226052064_110000/LConn3 -- T_226054226_110000;10000_ПС_110_10_кВ_Кибечи/LConn3 -- _CN_226054226_110000_CN_243069892_110000/LConn3 -- _CN_226054226_110000_CN_121218185_110000/RConn3 -- _CN_226054226_110000_CN_53366641_110000/RConn3 -- bus93/LConn1
  T_226052064_110000;10000_ПС_110_10_кВ_Шоркистры/LConn1 -- _CN_226054226_110000_CN_226052064_110000/RConn1
  T_226052064_110000;10000_ПС_110_10_кВ_Шоркистры/LConn2 -- _CN_226054226_110000_CN_226052064_110000/RConn2
  _CN_226054226_110000_CN_226052064_110000/RConn3 -- T_226052064_110000;10000_ПС_110_10_кВ_Шоркистры/LConn3 -- bus94/LConn1
  T_243069892_110000;35000;10000_ПС_110_35_10_кВ_Урмары/LConn1 -- _CN_226054226_110000_CN_243069892_110000/RConn1
  T_243069892_110000;35000;10000_ПС_110_35_10_кВ_Урмары/LConn2 -- _CN_226054226_110000_CN_243069892_110000/RConn2
  _CN_226054226_110000_CN_243069892_110000/RConn3 -- T_243069892_110000;35000;10000_ПС_110_35_10_кВ_Урмары/LConn3 -- bus95/LConn1
  _CN_279978581_110000_CN_219889824_110000/RConn1 -- T_279978581_110000;10000_ПС_110_10_кВ_Кувакино/LConn1 -- _CN_279978581_110000_CN_222133214_110000/LConn1 -- _CN_279978581_110000_CN_279978582_110000/RConn1
  _CN_279978581_110000_CN_219889824_110000/RConn2 -- T_279978581_110000;10000_ПС_110_10_кВ_Кувакино/LConn2 -- _CN_279978581_110000_CN_222133214_110000/LConn2 -- _CN_279978581_110000_CN_279978582_110000/RConn2
  _CN_279978581_110000_CN_219889824_110000/RConn3 -- T_279978581_110000;10000_ПС_110_10_кВ_Кувакино/LConn3 -- _CN_279978581_110000_CN_222133214_110000/LConn3 -- _CN_279978581_110000_CN_279978582_110000/RConn3 -- bus96/LConn1
  T_222133214_110000;10000_ПС_110_10_кВ_Семеновская/LConn1 -- _CN_279978581_110000_CN_222133214_110000/RConn1
  T_222133214_110000;10000_ПС_110_10_кВ_Семеновская/LConn2 -- _CN_279978581_110000_CN_222133214_110000/RConn2
  _CN_279978581_110000_CN_222133214_110000/RConn3 -- T_222133214_110000;10000_ПС_110_10_кВ_Семеновская/LConn3 -- bus97/LConn1
  _CN_108403292_110000_CN_62191058_110000/LConn1 -- T_108403292__/LConn1 -- _CN_108403292_110000_CN_94214974_110000/LConn1
  _CN_108403292_110000_CN_62191058_110000/LConn2 -- T_108403292__/LConn2 -- _CN_108403292_110000_CN_94214974_110000/LConn2
  _CN_108403292_110000_CN_62191058_110000/LConn3 -- T_108403292__/LConn3 -- _CN_108403292_110000_CN_94214974_110000/LConn3 -- bus98/LConn1
  G_62191058_Татарская_АЭС/RConn1 -- _CN_108403292_110000_CN_62191058_110000/RConn1
  G_62191058_Татарская_АЭС/RConn2 -- _CN_108403292_110000_CN_62191058_110000/RConn2
  _CN_108403292_110000_CN_62191058_110000/RConn3 -- G_62191058_Татарская_АЭС/RConn3 -- bus99/LConn1
  _CN_108403292_110000_CN_94214974_110000/RConn1 -- T_94214974__ПС_Нижнекамская/RConn1 -- _CN_94214974_110000_CN_104227390_110000/LConn1 -- L_94214974/LConn1
  _CN_108403292_110000_CN_94214974_110000/RConn2 -- T_94214974__ПС_Нижнекамская/RConn2 -- _CN_94214974_110000_CN_104227390_110000/LConn2 -- L_94214974/LConn2
  _CN_108403292_110000_CN_94214974_110000/RConn3 -- T_94214974__ПС_Нижнекамская/RConn3 -- _CN_94214974_110000_CN_104227390_110000/LConn3 -- L_94214974/LConn3 -- bus100/LConn1
  T_193928464__ПС_КПД/LConn1 -- _CN_193928464_110000_CN_109525418_110000/RConn1
  T_193928464__ПС_КПД/LConn2 -- _CN_193928464_110000_CN_109525418_110000/RConn2
  _CN_193928464_110000_CN_109525418_110000/RConn3 -- T_193928464__ПС_КПД/LConn3 -- bus101/LConn1
  T_102447718__/LConn1 -- _CN_102447718_110000_CN_308883878_110000/LConn1
  T_102447718__/LConn2 -- _CN_102447718_110000_CN_308883878_110000/LConn2
  _CN_102447718_110000_CN_308883878_110000/LConn3 -- T_102447718__/LConn3 -- bus102/LConn1
  T_308883878__/LConn1 -- _CN_102447718_110000_CN_308883878_110000/RConn1
  T_308883878__/LConn2 -- _CN_102447718_110000_CN_308883878_110000/RConn2
  _CN_102447718_110000_CN_308883878_110000/RConn3 -- T_308883878__/LConn3 -- bus103/LConn1
  _CN_279258960_110000_CN_241262030_110000/LConn1 -- T_279258960_110000;35000;10000_ПС_110_35_10_кВ_Красноармейская/LConn1 -- _CN_279258960_110000_CN_242972920_110000/RConn1 -- _CN_279258960_110000_CN_242932802_110000/LConn1
  _CN_279258960_110000_CN_241262030_110000/LConn2 -- T_279258960_110000;35000;10000_ПС_110_35_10_кВ_Красноармейская/LConn2 -- _CN_279258960_110000_CN_242972920_110000/RConn2 -- _CN_279258960_110000_CN_242932802_110000/LConn2
  _CN_279258960_110000_CN_241262030_110000/LConn3 -- T_279258960_110000;35000;10000_ПС_110_35_10_кВ_Красноармейская/LConn3 -- _CN_279258960_110000_CN_242972920_110000/RConn3 -- bus104/LConn1 -- _CN_279258960_110000_CN_242932802_110000/LConn3
  T_241262030_110000;35000;10000_ПС_110_35_10_кВ_Цивильск/LConn1 -- _CN_279258960_110000_CN_241262030_110000/RConn1
  T_241262030_110000;35000;10000_ПС_110_35_10_кВ_Цивильск/LConn2 -- _CN_279258960_110000_CN_241262030_110000/RConn2
  _CN_279258960_110000_CN_241262030_110000/RConn3 -- T_241262030_110000;35000;10000_ПС_110_35_10_кВ_Цивильск/LConn3 -- bus105/LConn1
  T_242932802_110000;10000_ПС_110_10_кВ_Оросительная/LConn1 -- _CN_279258960_110000_CN_242932802_110000/RConn1
  T_242932802_110000;10000_ПС_110_10_кВ_Оросительная/LConn2 -- _CN_279258960_110000_CN_242932802_110000/RConn2
  _CN_279258960_110000_CN_242932802_110000/RConn3 -- T_242932802_110000;10000_ПС_110_10_кВ_Оросительная/LConn3 -- bus106/LConn1
  ТЭЦ2_Кожино_110кВ_CN_110255218_110000_CN_107881747_110000/RConn1 -- T_110255218__ПС_Кожино_110_35кВ/LConn1 -- ТЭЦ2_Кожино_110кВ_CN_110255218_110000_CN_107692183_110000/LConn1
  ТЭЦ2_Кожино_110кВ_CN_110255218_110000_CN_107881747_110000/RConn2 -- T_110255218__ПС_Кожино_110_35кВ/LConn2 -- ТЭЦ2_Кожино_110кВ_CN_110255218_110000_CN_107692183_110000/LConn2
  ТЭЦ2_Кожино_110кВ_CN_110255218_110000_CN_107881747_110000/RConn3 -- T_110255218__ПС_Кожино_110_35кВ/LConn3 -- ТЭЦ2_Кожино_110кВ_CN_110255218_110000_CN_107692183_110000/LConn3 -- bus107/LConn1
  ТЭЦ2_Кожино_110кВ_CN_110255218_110000_CN_107692183_110000/RConn1 -- T_107692183_220000_ПС_Чигашево_220_110кВ/RConn1 -- _CN_107692183_110000_CN_107943661_110000/LConn1 -- _CN_107692183_110000_CN_107881747_110000/RConn1 -- L_107692183/LConn1
  ТЭЦ2_Кожино_110кВ_CN_110255218_110000_CN_107692183_110000/RConn2 -- T_107692183_220000_ПС_Чигашево_220_110кВ/RConn2 -- _CN_107692183_110000_CN_107943661_110000/LConn2 -- _CN_107692183_110000_CN_107881747_110000/RConn2 -- L_107692183/LConn2
  ТЭЦ2_Кожино_110кВ_CN_110255218_110000_CN_107692183_110000/RConn3 -- T_107692183_220000_ПС_Чигашево_220_110кВ/RConn3 -- _CN_107692183_110000_CN_107943661_110000/LConn3 -- _CN_107692183_110000_CN_107881747_110000/RConn3 -- L_107692183/LConn3 -- bus108/LConn1
  T_330006647_110000_/LConn1 -- _CN_330006647_110000_CN_116695201_110000/RConn1
  T_330006647_110000_/LConn2 -- _CN_330006647_110000_CN_116695201_110000/RConn2
  _CN_330006647_110000_CN_116695201_110000/RConn3 -- T_330006647_110000_/LConn3 -- bus109/LConn1
  _CN_57948286_110000_CN_51711248_110000/LConn1 -- T_57948286_110000;10000_Сазанлей/LConn1 -- _CN_57948286_110000_CN_51601242_110000/LConn1
  _CN_57948286_110000_CN_51711248_110000/LConn2 -- T_57948286_110000;10000_Сазанлей/LConn2 -- _CN_57948286_110000_CN_51601242_110000/LConn2
  _CN_57948286_110000_CN_51711248_110000/LConn3 -- T_57948286_110000;10000_Сазанлей/LConn3 -- _CN_57948286_110000_CN_51601242_110000/LConn3 -- bus110/LConn1
  T_51711248_110000_/LConn1 -- _CN_57948286_110000_CN_51711248_110000/RConn1
  T_51711248_110000_/LConn2 -- _CN_57948286_110000_CN_51711248_110000/RConn2
  _CN_57948286_110000_CN_51711248_110000/RConn3 -- T_51711248_110000_/LConn3 -- bus111/LConn1
  "T_51601242_220000;110000;fixme_ПС_220_кВ_\"Центральная\""/LConn1 -- _CN_57948286_110000_CN_51601242_110000/RConn1
  "T_51601242_220000;110000;fixme_ПС_220_кВ_\"Центральная\""/LConn2 -- _CN_57948286_110000_CN_51601242_110000/RConn2
  _CN_57948286_110000_CN_51601242_110000/RConn3 -- "T_51601242_220000;110000;fixme_ПС_220_кВ_\"Центральная\""/LConn3 -- bus112/LConn1
  _CN_244847744_110000_CN_279846258_110000/LConn1 -- T_244847744__/LConn1 -- _CN_244847744_110000_CN_280247940_110000/LConn1 -- _CN_244847744_110000_CN_280247942_110000/LConn1 -- _CN_244847744_110000_CN_207204995_110000/RConn1 -- _CN_244847744_110000_CN_280247938_110000/LConn1 -- _CN_244847744_110000_CN_53366641_110000/RConn1
  _CN_244847744_110000_CN_279846258_110000/LConn2 -- T_244847744__/LConn2 -- _CN_244847744_110000_CN_280247940_110000/LConn2 -- _CN_244847744_110000_CN_280247942_110000/LConn2 -- _CN_244847744_110000_CN_207204995_110000/RConn2 -- _CN_244847744_110000_CN_280247938_110000/LConn2 -- _CN_244847744_110000_CN_53366641_110000/RConn2
  _CN_244847744_110000_CN_279846258_110000/LConn3 -- T_244847744__/LConn3 -- _CN_244847744_110000_CN_280247940_110000/LConn3 -- _CN_244847744_110000_CN_280247942_110000/LConn3 -- _CN_244847744_110000_CN_207204995_110000/RConn3 -- _CN_244847744_110000_CN_280247938_110000/LConn3 -- _CN_244847744_110000_CN_53366641_110000/RConn3 -- bus113/LConn1
  T_279846258_110000;10000_ПС_110_10_кВ_Ачаксы/LConn1 -- _CN_244847744_110000_CN_279846258_110000/RConn1
  T_279846258_110000;10000_ПС_110_10_кВ_Ачаксы/LConn2 -- _CN_244847744_110000_CN_279846258_110000/RConn2
  _CN_244847744_110000_CN_279846258_110000/RConn3 -- T_279846258_110000;10000_ПС_110_10_кВ_Ачаксы/LConn3 -- bus114/LConn1
  T_280247940_110000;10000_ПС_110_10_кВ_Саланчики/LConn1 -- _CN_244847744_110000_CN_280247940_110000/RConn1
  T_280247940_110000;10000_ПС_110_10_кВ_Саланчики/LConn2 -- _CN_244847744_110000_CN_280247940_110000/RConn2
  _CN_244847744_110000_CN_280247940_110000/RConn3 -- T_280247940_110000;10000_ПС_110_10_кВ_Саланчики/LConn3 -- bus115/LConn1
  _CN_244847744_110000_CN_280247942_110000/RConn1 -- T_280247942_110000;35000;10000_ПС_110_35_10_кВ_Красночетайская/LConn1 -- _CN_280247955_110000_CN_280247942_110000/LConn1
  _CN_244847744_110000_CN_280247942_110000/RConn2 -- T_280247942_110000;35000;10000_ПС_110_35_10_кВ_Красночетайская/LConn2 -- _CN_280247955_110000_CN_280247942_110000/LConn2
  _CN_244847744_110000_CN_280247942_110000/RConn3 -- T_280247942_110000;35000;10000_ПС_110_35_10_кВ_Красночетайская/LConn3 -- _CN_280247955_110000_CN_280247942_110000/LConn3 -- bus116/LConn1
  T_280247938__/LConn1 -- _CN_244847744_110000_CN_280247938_110000/RConn1
  T_280247938__/LConn2 -- _CN_244847744_110000_CN_280247938_110000/RConn2
  _CN_244847744_110000_CN_280247938_110000/RConn3 -- T_280247938__/LConn3 -- bus117/LConn1
  T_207206840__Тяговая_подстанция/LConn1 -- _CN_207204995_110000_CN_207206840_110000/RConn1
  T_207206840__Тяговая_подстанция/LConn2 -- _CN_207204995_110000_CN_207206840_110000/RConn2
  _CN_207204995_110000_CN_207206840_110000/RConn3 -- T_207206840__Тяговая_подстанция/LConn3 -- bus118/LConn1
  "T_56048772_220000_Электрическая_подстанция_\"Горная\""/LConn1 -- _CN_56048772_110000_CN_53566695_110000/LConn1
  "T_56048772_220000_Электрическая_подстанция_\"Горная\""/LConn2 -- _CN_56048772_110000_CN_53566695_110000/LConn2
  _CN_56048772_110000_CN_53566695_110000/LConn3 -- "T_56048772_220000_Электрическая_подстанция_\"Горная\""/LConn3 -- bus119/LConn1
  T_53566695__Подстанция_Кизел_(ж_д)/LConn1 -- _CN_56048772_110000_CN_53566695_110000/RConn1
  T_53566695__Подстанция_Кизел_(ж_д)/LConn2 -- _CN_56048772_110000_CN_53566695_110000/RConn2
  _CN_56048772_110000_CN_53566695_110000/RConn3 -- T_53566695__Подстанция_Кизел_(ж_д)/LConn3 -- bus120/LConn1
  T_116695174_110000_ПС_110_6_кВ_Инструментальная/LConn1 -- _CN_116695174_110000_CN_283379848_110000/RConn1
  T_116695174_110000_ПС_110_6_кВ_Инструментальная/LConn2 -- _CN_116695174_110000_CN_283379848_110000/RConn2
  _CN_116695174_110000_CN_283379848_110000/RConn3 -- T_116695174_110000_ПС_110_6_кВ_Инструментальная/LConn3 -- bus121/LConn1
  T_191841753__ПС_Свияжск/LConn1 -- ВЛ_Свияжск___Тюрлема_110кВ_CN_121218185_110000_CN_191841753_110000/RConn1
  T_191841753__ПС_Свияжск/LConn2 -- ВЛ_Свияжск___Тюрлема_110кВ_CN_121218185_110000_CN_191841753_110000/RConn2
  ВЛ_Свияжск___Тюрлема_110кВ_CN_121218185_110000_CN_191841753_110000/RConn3 -- T_191841753__ПС_Свияжск/LConn3 -- bus122/LConn1
  T_226055643__/LConn1 -- _CN_121218185_110000_CN_226055643_110000/RConn1
  T_226055643__/LConn2 -- _CN_121218185_110000_CN_226055643_110000/RConn2
  _CN_121218185_110000_CN_226055643_110000/RConn3 -- T_226055643__/LConn3 -- bus123/LConn1
  T_280247955_110000;35000;10000_ПС_110_35_10_кВ_Кукшум/LConn1 -- _CN_280247955_110000_CN_280247942_110000/RConn1
  T_280247955_110000;35000;10000_ПС_110_35_10_кВ_Кукшум/LConn2 -- _CN_280247955_110000_CN_280247942_110000/RConn2
  _CN_280247955_110000_CN_280247942_110000/RConn3 -- T_280247955_110000;35000;10000_ПС_110_35_10_кВ_Кукшум/LConn3 -- bus124/LConn1
  T_280247957_110000;35000;10000_ПС_110_35_10_кВ_ЯМЗ/LConn1 -- _CN_280247957_110000_CN_315675920_110000/LConn1
  T_280247957_110000;35000;10000_ПС_110_35_10_кВ_ЯМЗ/LConn2 -- _CN_280247957_110000_CN_315675920_110000/LConn2
  _CN_280247957_110000_CN_315675920_110000/LConn3 -- T_280247957_110000;35000;10000_ПС_110_35_10_кВ_ЯМЗ/LConn3 -- bus125/LConn1
  T_315675920_110000;10000_ПС_Покров_Майдан_110_10_кВ/LConn1 -- _CN_280247957_110000_CN_315675920_110000/RConn1
  T_315675920_110000;10000_ПС_Покров_Майдан_110_10_кВ/LConn2 -- _CN_280247957_110000_CN_315675920_110000/RConn2
  _CN_280247957_110000_CN_315675920_110000/RConn3 -- T_315675920_110000;10000_ПС_Покров_Майдан_110_10_кВ/LConn3 -- bus126/LConn1
  _CN_107692183_110000_CN_107943661_110000/RConn1 -- T_107943661_110000_Медведевский_электроучасток/LConn1 -- Медвед__Красноокт__110кВ_CN_110370987_110000_CN_107943661_110000/LConn1
  _CN_107692183_110000_CN_107943661_110000/RConn2 -- T_107943661_110000_Медведевский_электроучасток/LConn2 -- Медвед__Красноокт__110кВ_CN_110370987_110000_CN_107943661_110000/LConn2
  _CN_107692183_110000_CN_107943661_110000/RConn3 -- T_107943661_110000_Медведевский_электроучасток/LConn3 -- Медвед__Красноокт__110кВ_CN_110370987_110000_CN_107943661_110000/LConn3 -- bus127/LConn1
  T_176859804__Жасминная/LConn1 -- _CN_176859804_110000_CN_176642248_110000/LConn1
  T_176859804__Жасминная/LConn2 -- _CN_176859804_110000_CN_176642248_110000/LConn2
  _CN_176859804_110000_CN_176642248_110000/LConn3 -- T_176859804__Жасминная/LConn3 -- bus128/LConn1
  T_176642248__Елшанка_2/LConn1 -- _CN_176859804_110000_CN_176642248_110000/RConn1
  T_176642248__Елшанка_2/LConn2 -- _CN_176859804_110000_CN_176642248_110000/RConn2
  _CN_176859804_110000_CN_176642248_110000/RConn3 -- T_176642248__Елшанка_2/LConn3 -- bus129/LConn1
  T_243531233__ПС_Малмыж/LConn1 -- ВЛ_Вятские_Поляны___Малмыж_110кВ_CN_243531233_110000_CN_247403714_110000/LConn1
  T_243531233__ПС_Малмыж/LConn2 -- ВЛ_Вятские_Поляны___Малмыж_110кВ_CN_243531233_110000_CN_247403714_110000/LConn2
  ВЛ_Вятские_Поляны___Малмыж_110кВ_CN_243531233_110000_CN_247403714_110000/LConn3 -- T_243531233__ПС_Малмыж/LConn3 -- bus130/LConn1
  T_247403714__ПС_Сардек/LConn1 -- ВЛ_Вятские_Поляны___Малмыж_110кВ_CN_243531233_110000_CN_247403714_110000/RConn1
  T_247403714__ПС_Сардек/LConn2 -- ВЛ_Вятские_Поляны___Малмыж_110кВ_CN_243531233_110000_CN_247403714_110000/RConn2
  ВЛ_Вятские_Поляны___Малмыж_110кВ_CN_243531233_110000_CN_247403714_110000/RConn3 -- T_247403714__ПС_Сардек/LConn3 -- bus131/LConn1
  Медвед__Красноокт__110кВ_CN_110370987_110000_CN_107943661_110000/RConn1 -- T_110370987__ПС_Краснооктябрьск_110_10кВ/LConn1 -- Медвед__Красноокт__110кВ_CN_110370987_110000_CN_112681450_110000/LConn1
  Медвед__Красноокт__110кВ_CN_110370987_110000_CN_107943661_110000/RConn2 -- T_110370987__ПС_Краснооктябрьск_110_10кВ/LConn2 -- Медвед__Красноокт__110кВ_CN_110370987_110000_CN_112681450_110000/LConn2
  Медвед__Красноокт__110кВ_CN_110370987_110000_CN_107943661_110000/RConn3 -- T_110370987__ПС_Краснооктябрьск_110_10кВ/LConn3 -- Медвед__Красноокт__110кВ_CN_110370987_110000_CN_112681450_110000/LConn3 -- bus132/LConn1
  T_112681450_110000_/LConn1 -- Медвед__Красноокт__110кВ_CN_110370987_110000_CN_112681450_110000/RConn1
  T_112681450_110000_/LConn2 -- Медвед__Красноокт__110кВ_CN_110370987_110000_CN_112681450_110000/RConn2
  Медвед__Красноокт__110кВ_CN_110370987_110000_CN_112681450_110000/RConn3 -- T_112681450_110000_/LConn3 -- bus133/LConn1
  T_319459210__/LConn1 -- _CN_319459210_110000_CN_319459220_110000/LConn1
  T_319459210__/LConn2 -- _CN_319459210_110000_CN_319459220_110000/LConn2
  _CN_319459210_110000_CN_319459220_110000/LConn3 -- T_319459210__/LConn3 -- bus134/LConn1
  T_319459220_110000;10000_Перемская/LConn1 -- _CN_319459210_110000_CN_319459220_110000/RConn1
  T_319459220_110000;10000_Перемская/LConn2 -- _CN_319459210_110000_CN_319459220_110000/RConn2
  _CN_319459210_110000_CN_319459220_110000/RConn3 -- T_319459220_110000;10000_Перемская/LConn3 -- bus135/LConn1
  _CN_243154612_110000_CN_243820930_110000/LConn1 -- T_243154612__/LConn1 -- _CN_243154612_110000_CN_53366641_110000/RConn1
  _CN_243154612_110000_CN_243820930_110000/LConn2 -- T_243154612__/LConn2 -- _CN_243154612_110000_CN_53366641_110000/RConn2
  _CN_243154612_110000_CN_243820930_110000/LConn3 -- T_243154612__/LConn3 -- _CN_243154612_110000_CN_53366641_110000/RConn3 -- bus136/LConn1
  T_243820930__/LConn1 -- _CN_243154612_110000_CN_243820930_110000/RConn1
  T_243820930__/LConn2 -- _CN_243154612_110000_CN_243820930_110000/RConn2
  _CN_243154612_110000_CN_243820930_110000/RConn3 -- T_243820930__/LConn3 -- bus137/LConn1
  T_97060032__/LConn1 -- _CN_97060032_110000_CN_109525418_110000/RConn1
  T_97060032__/LConn2 -- _CN_97060032_110000_CN_109525418_110000/RConn2
  _CN_97060032_110000_CN_109525418_110000/RConn3 -- T_97060032__/LConn3 -- bus138/LConn1
  _CN_97060037_110000_CN_109525418_110000/RConn1 -- T_97060037__/LConn1 -- _CN_97060037_110000_CN_100584516_110000/LConn1
  _CN_97060037_110000_CN_109525418_110000/RConn2 -- T_97060037__/LConn2 -- _CN_97060037_110000_CN_100584516_110000/LConn2
  _CN_97060037_110000_CN_109525418_110000/RConn3 -- T_97060037__/LConn3 -- _CN_97060037_110000_CN_100584516_110000/LConn3 -- bus139/LConn1
  T_100584516__/LConn1 -- _CN_97060037_110000_CN_100584516_110000/RConn1
  T_100584516__/LConn2 -- _CN_97060037_110000_CN_100584516_110000/RConn2
  _CN_97060037_110000_CN_100584516_110000/RConn3 -- T_100584516__/LConn3 -- bus140/LConn1
  "T_327245366_110000_ПС_110_10кВ_\"Разино\""/LConn1 -- _CN_327245366_110000_CN_305832833_110000/LConn1
  "T_327245366_110000_ПС_110_10кВ_\"Разино\""/LConn2 -- _CN_327245366_110000_CN_305832833_110000/LConn2
  _CN_327245366_110000_CN_305832833_110000/LConn3 -- "T_327245366_110000_ПС_110_10кВ_\"Разино\""/LConn3 -- bus141/LConn1
  _CN_327245366_110000_CN_305832833_110000/RConn1 -- "T_305832833_110000_ПС_110_10кВ_\"Мадаево\""/LConn1 -- _CN_305832833_110000_CN_327245371_110000/LConn1
  _CN_327245366_110000_CN_305832833_110000/RConn2 -- "T_305832833_110000_ПС_110_10кВ_\"Мадаево\""/LConn2 -- _CN_305832833_110000_CN_327245371_110000/LConn2
  _CN_327245366_110000_CN_305832833_110000/RConn3 -- "T_305832833_110000_ПС_110_10кВ_\"Мадаево\""/LConn3 -- _CN_305832833_110000_CN_327245371_110000/LConn3 -- bus142/LConn1
  T_106289362__/LConn1 -- _CN_106289362_110000_CN_106289442_110000/LConn1
  T_106289362__/LConn2 -- _CN_106289362_110000_CN_106289442_110000/LConn2
  _CN_106289362_110000_CN_106289442_110000/LConn3 -- T_106289362__/LConn3 -- bus143/LConn1
  T_106289442__/LConn1 -- _CN_106289362_110000_CN_106289442_110000/RConn1
  T_106289442__/LConn2 -- _CN_106289362_110000_CN_106289442_110000/RConn2
  _CN_106289362_110000_CN_106289442_110000/RConn3 -- T_106289442__/LConn3 -- bus144/LConn1
  T_55334100__/LConn1 -- _CN_55334100_110000_CN_55334115_110000/LConn1
  T_55334100__/LConn2 -- _CN_55334100_110000_CN_55334115_110000/LConn2
  _CN_55334100_110000_CN_55334115_110000/LConn3 -- T_55334100__/LConn3 -- bus145/LConn1
  T_55334115__/LConn1 -- _CN_55334100_110000_CN_55334115_110000/RConn1
  T_55334115__/LConn2 -- _CN_55334100_110000_CN_55334115_110000/RConn2
  _CN_55334100_110000_CN_55334115_110000/RConn3 -- T_55334115__/LConn3 -- bus146/LConn1
  "T_327245584_110000_ПС_110_10кВ_\"Лукоянов_110\""/LConn1 -- _CN_327245584_110000_CN_327245371_110000/LConn1
  "T_327245584_110000_ПС_110_10кВ_\"Лукоянов_110\""/LConn2 -- _CN_327245584_110000_CN_327245371_110000/LConn2
  _CN_327245584_110000_CN_327245371_110000/LConn3 -- "T_327245584_110000_ПС_110_10кВ_\"Лукоянов_110\""/LConn3 -- bus147/LConn1
  _CN_327245584_110000_CN_327245371_110000/RConn1 -- "T_327245371_110000_ПС_110_35_10кВ_\"Починки_110\""/LConn1 -- _CN_305832833_110000_CN_327245371_110000/RConn1
  _CN_327245584_110000_CN_327245371_110000/RConn2 -- "T_327245371_110000_ПС_110_35_10кВ_\"Починки_110\""/LConn2 -- _CN_305832833_110000_CN_327245371_110000/RConn2
  _CN_327245584_110000_CN_327245371_110000/RConn3 -- "T_327245371_110000_ПС_110_35_10кВ_\"Починки_110\""/LConn3 -- _CN_305832833_110000_CN_327245371_110000/RConn3 -- bus148/LConn1
  T_58880346_110000;35000;10000_ПС_110_35_10_кВ_Спутник/LConn1 -- _CN_313773131_110000_CN_58880346_110000/RConn1
  T_58880346_110000;35000;10000_ПС_110_35_10_кВ_Спутник/LConn2 -- _CN_313773131_110000_CN_58880346_110000/RConn2
  _CN_313773131_110000_CN_58880346_110000/RConn3 -- T_58880346_110000;35000;10000_ПС_110_35_10_кВ_Спутник/LConn3 -- bus149/LConn1
  T_281879365_110000;10000_ПС_110_10_кВ_Светлая/LConn1 -- _CN_313773131_110000_CN_281879365_110000/RConn1
  T_281879365_110000;10000_ПС_110_10_кВ_Светлая/LConn2 -- _CN_313773131_110000_CN_281879365_110000/RConn2
  _CN_313773131_110000_CN_281879365_110000/RConn3 -- T_281879365_110000;10000_ПС_110_10_кВ_Светлая/LConn3 -- bus150/LConn1
  T_337947383__/LConn1 -- _CN_337947383_110000_CN_220103258_110000/LConn1
  T_337947383__/LConn2 -- _CN_337947383_110000_CN_220103258_110000/LConn2
  _CN_337947383_110000_CN_220103258_110000/LConn3 -- T_337947383__/LConn3 -- bus151/LConn1
  G_220103258_Зауральская_ТЭЦ/RConn1 -- _CN_337947383_110000_CN_220103258_110000/RConn1
  G_220103258_Зауральская_ТЭЦ/RConn2 -- _CN_337947383_110000_CN_220103258_110000/RConn2
  _CN_337947383_110000_CN_220103258_110000/RConn3 -- G_220103258_Зауральская_ТЭЦ/RConn3 -- bus152/LConn1
  T_90868997__/LConn1 -- _CN_90868997_110000_CN_67498838_110000/RConn1
  T_90868997__/LConn2 -- _CN_90868997_110000_CN_67498838_110000/RConn2
  _CN_90868997_110000_CN_67498838_110000/RConn3 -- T_90868997__/LConn3 -- bus153/LConn1
  _CN_211578632_110000_CN_307428692_110000/LConn1 -- T_211578632_110000_ПС_СИЛЬВИНИТ/LConn1 -- _CN_211578632_110000_CN_245404985_110000/LConn1
  _CN_211578632_110000_CN_307428692_110000/LConn2 -- T_211578632_110000_ПС_СИЛЬВИНИТ/LConn2 -- _CN_211578632_110000_CN_245404985_110000/LConn2
  _CN_211578632_110000_CN_307428692_110000/LConn3 -- T_211578632_110000_ПС_СИЛЬВИНИТ/LConn3 -- _CN_211578632_110000_CN_245404985_110000/LConn3 -- bus154/LConn1
  T_307428692__Сибирь/LConn1 -- _CN_211578632_110000_CN_307428692_110000/RConn1
  T_307428692__Сибирь/LConn2 -- _CN_211578632_110000_CN_307428692_110000/RConn2
  _CN_211578632_110000_CN_307428692_110000/RConn3 -- T_307428692__Сибирь/LConn3 -- bus155/LConn1
  T_245404985_110000_ПС_Уньва/LConn1 -- _CN_211578632_110000_CN_245404985_110000/RConn1
  T_245404985_110000_ПС_Уньва/LConn2 -- _CN_211578632_110000_CN_245404985_110000/RConn2
  _CN_211578632_110000_CN_245404985_110000/RConn3 -- T_245404985_110000_ПС_Уньва/LConn3 -- bus156/LConn1
  T_286921936__/LConn1 -- _CN_286921936_110000_CN_109525394_110000/LConn1
  T_286921936__/LConn2 -- _CN_286921936_110000_CN_109525394_110000/LConn2
  _CN_286921936_110000_CN_109525394_110000/LConn3 -- T_286921936__/LConn3 -- bus157/LConn1
  _CN_286921936_110000_CN_109525394_110000/RConn1 -- T_109525394_220000_ПС_220_кВ_Калийная/LConn1 -- _CN_109525394_110000_CN_109525404_110000/LConn1 -- _CN_109525394_110000_CN_109525439_110000/LConn1
  _CN_286921936_110000_CN_109525394_110000/RConn2 -- T_109525394_220000_ПС_220_кВ_Калийная/LConn2 -- _CN_109525394_110000_CN_109525404_110000/LConn2 -- _CN_109525394_110000_CN_109525439_110000/LConn2
  _CN_286921936_110000_CN_109525394_110000/RConn3 -- T_109525394_220000_ПС_220_кВ_Калийная/LConn3 -- _CN_109525394_110000_CN_109525404_110000/LConn3 -- bus158/LConn1 -- _CN_109525394_110000_CN_109525439_110000/LConn3
  T_103877395__/LConn1 -- _CN_103877395_110000_CN_103877470_110000/LConn1
  T_103877395__/LConn2 -- _CN_103877395_110000_CN_103877470_110000/LConn2
  _CN_103877395_110000_CN_103877470_110000/LConn3 -- T_103877395__/LConn3 -- bus159/LConn1
  T_103877470__/LConn1 -- _CN_103877395_110000_CN_103877470_110000/RConn1
  T_103877470__/LConn2 -- _CN_103877395_110000_CN_103877470_110000/RConn2
  _CN_103877395_110000_CN_103877470_110000/RConn3 -- T_103877470__/LConn3 -- bus160/LConn1
  T_287462706_110000_110_КВ_Тёплая_Гора/LConn1 -- _CN_287462706_110000_CN_238317576_110000/LConn1
  T_287462706_110000_110_КВ_Тёплая_Гора/LConn2 -- _CN_287462706_110000_CN_238317576_110000/LConn2
  _CN_287462706_110000_CN_238317576_110000/LConn3 -- T_287462706_110000_110_КВ_Тёплая_Гора/LConn3 -- bus161/LConn1
  T_238317576__/LConn1 -- _CN_287462706_110000_CN_238317576_110000/RConn1
  T_238317576__/LConn2 -- _CN_287462706_110000_CN_238317576_110000/RConn2
  _CN_287462706_110000_CN_238317576_110000/RConn3 -- T_238317576__/LConn3 -- bus162/LConn1
  T_252815158_110000;35000;10000_/LConn1 -- _CN_252815158_110000_CN_252815157_110000/LConn1
  T_252815158_110000;35000;10000_/LConn2 -- _CN_252815158_110000_CN_252815157_110000/LConn2
  _CN_252815158_110000_CN_252815157_110000/LConn3 -- T_252815158_110000;35000;10000_/LConn3 -- bus163/LConn1
  T_252815157__/LConn1 -- _CN_252815158_110000_CN_252815157_110000/RConn1
  T_252815157__/LConn2 -- _CN_252815158_110000_CN_252815157_110000/RConn2
  _CN_252815158_110000_CN_252815157_110000/RConn3 -- T_252815157__/LConn3 -- bus164/LConn1
  T_290776375_110000_ПС_ЗАГОТОВКА/LConn1 -- _CN_290776375_110000_CN_290777752_110000/LConn1
  T_290776375_110000_ПС_ЗАГОТОВКА/LConn2 -- _CN_290776375_110000_CN_290777752_110000/LConn2
  _CN_290776375_110000_CN_290777752_110000/LConn3 -- T_290776375_110000_ПС_ЗАГОТОВКА/LConn3 -- bus165/LConn1
  T_290777752_110000_ГРЕМЯЧАЯ_I/LConn1 -- _CN_290776375_110000_CN_290777752_110000/RConn1
  T_290777752_110000_ГРЕМЯЧАЯ_I/LConn2 -- _CN_290776375_110000_CN_290777752_110000/RConn2
  _CN_290776375_110000_CN_290777752_110000/RConn3 -- T_290777752_110000_ГРЕМЯЧАЯ_I/LConn3 -- bus166/LConn1
  G_104227390_ТЭЦ_2/RConn1 -- _CN_94214974_110000_CN_104227390_110000/RConn1
  G_104227390_ТЭЦ_2/RConn2 -- _CN_94214974_110000_CN_104227390_110000/RConn2
  _CN_94214974_110000_CN_104227390_110000/RConn3 -- G_104227390_ТЭЦ_2/RConn3 -- bus167/LConn1
  T_93482493__/LConn1 -- _CN_67498838_110000_CN_93482493_110000/RConn1
  T_93482493__/LConn2 -- _CN_67498838_110000_CN_93482493_110000/RConn2
  _CN_67498838_110000_CN_93482493_110000/RConn3 -- T_93482493__/LConn3 -- bus168/LConn1
  T_242610017_110000;35000;10000_ПС_110_35_10_кВ_Лесная/LConn1 -- "110_кВ_\"Лесная_Тормозная\"_CN_242610017_110000_CN_242614771_110000"/LConn1
  T_242610017_110000;35000;10000_ПС_110_35_10_кВ_Лесная/LConn2 -- "110_кВ_\"Лесная_Тормозная\"_CN_242610017_110000_CN_242614771_110000"/LConn2
  "110_кВ_\"Лесная_Тормозная\"_CN_242610017_110000_CN_242614771_110000"/LConn3 -- T_242610017_110000;35000;10000_ПС_110_35_10_кВ_Лесная/LConn3 -- bus169/LConn1
  T_242614771_110000;6000_ПС_110_6_кВ_Тормозная/LConn1 -- "110_кВ_\"Лесная_Тормозная\"_CN_242610017_110000_CN_242614771_110000"/RConn1
  T_242614771_110000;6000_ПС_110_6_кВ_Тормозная/LConn2 -- "110_кВ_\"Лесная_Тормозная\"_CN_242610017_110000_CN_242614771_110000"/RConn2
  "110_кВ_\"Лесная_Тормозная\"_CN_242610017_110000_CN_242614771_110000"/RConn3 -- T_242614771_110000;6000_ПС_110_6_кВ_Тормозная/LConn3 -- bus170/LConn1
  T_207740804_110000;10000_ПС_110_10_кВ_Дружба/LConn1 -- ВЛ_110_кВ_Канаш_Дружба_CN_53366641_110000_CN_207740804_110000/RConn1
  T_207740804_110000;10000_ПС_110_10_кВ_Дружба/LConn2 -- ВЛ_110_кВ_Канаш_Дружба_CN_53366641_110000_CN_207740804_110000/RConn2
  ВЛ_110_кВ_Канаш_Дружба_CN_53366641_110000_CN_207740804_110000/RConn3 -- T_207740804_110000;10000_ПС_110_10_кВ_Дружба/LConn3 -- bus171/LConn1
  T_279846262_110000;10000_ПС_110_10_кВ_Атнашево/LConn1 -- ВЛ_110_кВ_Канаш_Дружба_CN_53366641_110000_CN_279846262_110000/RConn1
  T_279846262_110000;10000_ПС_110_10_кВ_Атнашево/LConn2 -- ВЛ_110_кВ_Канаш_Дружба_CN_53366641_110000_CN_279846262_110000/RConn2
  ВЛ_110_кВ_Канаш_Дружба_CN_53366641_110000_CN_279846262_110000/RConn3 -- T_279846262_110000;10000_ПС_110_10_кВ_Атнашево/LConn3 -- bus172/LConn1
  T_113994637__ПС_Буинск/LConn1 -- _CN_113994637_110000_CN_171977680_110000/RConn1
  T_113994637__ПС_Буинск/LConn2 -- _CN_113994637_110000_CN_171977680_110000/RConn2
  _CN_113994637_110000_CN_171977680_110000/RConn3 -- T_113994637__ПС_Буинск/LConn3 -- bus173/LConn1
  T_109525439__/LConn1 -- _CN_109525394_110000_CN_109525439_110000/RConn1
  T_109525439__/LConn2 -- _CN_109525394_110000_CN_109525439_110000/RConn2
  _CN_109525394_110000_CN_109525439_110000/RConn3 -- T_109525439__/LConn3 -- bus174/LConn1
  T_109525404__/LConn1 -- _CN_109525394_110000_CN_109525404_110000/RConn1
  T_109525404__/LConn2 -- _CN_109525394_110000_CN_109525404_110000/RConn2
  _CN_109525394_110000_CN_109525404_110000/RConn3 -- T_109525404__/LConn3 -- bus175/LConn1
  T_172819864__Содовая_1_110_35_6/LConn1 -- _CN_172819864_110000_CN_109525418_110000/RConn1
  T_172819864__Содовая_1_110_35_6/LConn2 -- _CN_172819864_110000_CN_109525418_110000/RConn2
  _CN_172819864_110000_CN_109525418_110000/RConn3 -- T_172819864__Содовая_1_110_35_6/LConn3 -- bus176/LConn1
  T_190492574__/LConn1 -- _CN_190492574_110000_CN_108913072_110000/LConn1
  T_190492574__/LConn2 -- _CN_190492574_110000_CN_108913072_110000/LConn2
  _CN_190492574_110000_CN_108913072_110000/LConn3 -- T_190492574__/LConn3 -- bus177/LConn1
  T_108913072_110000;10000_Подстанция/LConn1 -- _CN_190492574_110000_CN_108913072_110000/RConn1
  T_108913072_110000;10000_Подстанция/LConn2 -- _CN_190492574_110000_CN_108913072_110000/RConn2
  _CN_190492574_110000_CN_108913072_110000/RConn3 -- T_108913072_110000;10000_Подстанция/LConn3 -- bus178/LConn1
  T_70186926_110000;fixme_Дубравная/LConn1 -- _CN_70186926_110000_CN_70186927_110000/LConn1
  T_70186926_110000;fixme_Дубравная/LConn2 -- _CN_70186926_110000_CN_70186927_110000/LConn2
  _CN_70186926_110000_CN_70186927_110000/LConn3 -- T_70186926_110000;fixme_Дубравная/LConn3 -- bus179/LConn1
  T_70186927_110000;fixme_ЗКПД/LConn1 -- _CN_70186926_110000_CN_70186927_110000/RConn1
  T_70186927_110000;fixme_ЗКПД/LConn2 -- _CN_70186926_110000_CN_70186927_110000/RConn2
  _CN_70186926_110000_CN_70186927_110000/RConn3 -- T_70186927_110000;fixme_ЗКПД/LConn3 -- bus180/LConn1
  T_136761822_110000_/LConn1 -- _CN_136761822_110000_CN_245072101_110000/LConn1
  T_136761822_110000_/LConn2 -- _CN_136761822_110000_CN_245072101_110000/LConn2
  _CN_136761822_110000_CN_245072101_110000/LConn3 -- T_136761822_110000_/LConn3 -- bus181/LConn1
  _CN_136761822_110000_CN_245072101_110000/RConn1 -- G_245072101_Жигулёвская_ГЭС/RConn1 -- _CN_110601218_500000_CN_245072101_110000/LConn1
  _CN_136761822_110000_CN_245072101_110000/RConn2 -- G_245072101_Жигулёвская_ГЭС/RConn2 -- _CN_110601218_500000_CN_245072101_110000/LConn2
  _CN_136761822_110000_CN_245072101_110000/RConn3 -- G_245072101_Жигулёвская_ГЭС/RConn3 -- _CN_110601218_500000_CN_245072101_110000/LConn3 -- bus182/LConn1
  Рузаевка___Мокша_CN_274998912_220000_CN_113585698_220000/LConn1 -- T_274998912_220000_Мокша/LConn1 -- Рузаевка___Мокша_CN_274998912_220000_CN_72288676_220000/LConn1
  Рузаевка___Мокша_CN_274998912_220000_CN_113585698_220000/LConn2 -- T_274998912_220000_Мокша/LConn2 -- Рузаевка___Мокша_CN_274998912_220000_CN_72288676_220000/LConn2
  Рузаевка___Мокша_CN_274998912_220000_CN_113585698_220000/LConn3 -- T_274998912_220000_Мокша/LConn3 -- Рузаевка___Мокша_CN_274998912_220000_CN_72288676_220000/LConn3 -- bus183/LConn1
  Рузаевка___Мокша_CN_274998912_220000_CN_113585698_220000/RConn1 -- T_113585698_220000_ПС_220кВ_Рузаевка/LConn1 -- Рузаевка___Центролит_CN_113585698_220000_CN_92419131_220000/LConn1 -- Рузаевка___Центролит_CN_113585698_220000_CN_327226015_220000/LConn1 -- Рузаевка___Центролит_CN_113585698_220000_CN_72288676_220000/LConn1 -- Рузаевка___Центролит_CN_113585698_220000_CN_103735794_220000/LConn1 -- Пенза_2___Рузаевка_CN_113585698_220000_CN_211405161_220000/LConn1
  Рузаевка___Мокша_CN_274998912_220000_CN_113585698_220000/RConn2 -- T_113585698_220000_ПС_220кВ_Рузаевка/LConn2 -- Рузаевка___Центролит_CN_113585698_220000_CN_92419131_220000/LConn2 -- Рузаевка___Центролит_CN_113585698_220000_CN_327226015_220000/LConn2 -- Рузаевка___Центролит_CN_113585698_220000_CN_72288676_220000/LConn2 -- Рузаевка___Центролит_CN_113585698_220000_CN_103735794_220000/LConn2 -- Пенза_2___Рузаевка_CN_113585698_220000_CN_211405161_220000/LConn2
  Рузаевка___Мокша_CN_274998912_220000_CN_113585698_220000/RConn3 -- T_113585698_220000_ПС_220кВ_Рузаевка/LConn3 -- Рузаевка___Центролит_CN_113585698_220000_CN_92419131_220000/LConn3 -- Рузаевка___Центролит_CN_113585698_220000_CN_327226015_220000/LConn3 -- Рузаевка___Центролит_CN_113585698_220000_CN_72288676_220000/LConn3 -- Рузаевка___Центролит_CN_113585698_220000_CN_103735794_220000/LConn3 -- Пенза_2___Рузаевка_CN_113585698_220000_CN_211405161_220000/LConn3 -- bus184/LConn1
  Рузаевка___Мокша_CN_274998912_220000_CN_72288676_220000/RConn1 -- T_72288676_500000_Арзамасская/RConn1 -- Арзамасская___Лукояновская_№1_CN_305832836_220000_CN_72288676_220000/LConn1 -- _CN_327325460_220000_CN_72288676_220000/LConn1 -- Рузаевка___Центролит_CN_113585698_220000_CN_72288676_220000/RConn1 -- Арзамасская_Сергач_CN_72288676_220000_CN_277905350_220000/LConn1 -- L_72288676/LConn1
  Рузаевка___Мокша_CN_274998912_220000_CN_72288676_220000/RConn2 -- T_72288676_500000_Арзамасская/RConn2 -- Арзамасская___Лукояновская_№1_CN_305832836_220000_CN_72288676_220000/LConn2 -- _CN_327325460_220000_CN_72288676_220000/LConn2 -- Рузаевка___Центролит_CN_113585698_220000_CN_72288676_220000/RConn2 -- Арзамасская_Сергач_CN_72288676_220000_CN_277905350_220000/LConn2 -- L_72288676/LConn2
  Рузаевка___Мокша_CN_274998912_220000_CN_72288676_220000/RConn3 -- T_72288676_500000_Арзамасская/RConn3 -- Арзамасская___Лукояновская_№1_CN_305832836_220000_CN_72288676_220000/LConn3 -- _CN_327325460_220000_CN_72288676_220000/LConn3 -- Рузаевка___Центролит_CN_113585698_220000_CN_72288676_220000/RConn3 -- Арзамасская_Сергач_CN_72288676_220000_CN_277905350_220000/LConn3 -- L_72288676/LConn3 -- bus185/LConn1
  T_327816066_220000_Кузнецк/LConn1 -- _CN_327816066_220000_CN_211405161_220000/LConn1
  T_327816066_220000_Кузнецк/LConn2 -- _CN_327816066_220000_CN_211405161_220000/LConn2
  _CN_327816066_220000_CN_211405161_220000/LConn3 -- T_327816066_220000_Кузнецк/LConn3 -- bus186/LConn1
  _CN_327816066_220000_CN_211405161_220000/RConn1 -- T_211405161_220000_Пенза_1/LConn1 -- Пенза_2___Рузаевка_CN_113585698_220000_CN_211405161_220000/RConn1
  _CN_327816066_220000_CN_211405161_220000/RConn2 -- T_211405161_220000_Пенза_1/LConn2 -- Пенза_2___Рузаевка_CN_113585698_220000_CN_211405161_220000/RConn2
  _CN_327816066_220000_CN_211405161_220000/RConn3 -- T_211405161_220000_Пенза_1/LConn3 -- Пенза_2___Рузаевка_CN_113585698_220000_CN_211405161_220000/RConn3 -- bus187/LConn1
  Чебоксарская_ГЭС___Венец_CN_207204995_220000_CN_305893253_220000/LConn1 -- T_207204995_220000;110000;6000_ПС_Венец_220_110_6_кВ/LConn1 -- Чебоксарская_ГЭС___Венец_CN_207204995_220000_CN_53366641_220000/LConn1 -- Чебоксарская_ГЭС___Венец_CN_207204995_220000_CN_121218185_220000/LConn1 -- Чебоксарская_ГЭС___Венец_CN_207204995_220000_CN_107692183_220000/LConn1 -- Чебоксарская_ГЭС___Венец_CN_207204995_220000_CN_93292147_220000/LConn1
  Чебоксарская_ГЭС___Венец_CN_207204995_220000_CN_305893253_220000/LConn2 -- T_207204995_220000;110000;6000_ПС_Венец_220_110_6_кВ/LConn2 -- Чебоксарская_ГЭС___Венец_CN_207204995_220000_CN_53366641_220000/LConn2 -- Чебоксарская_ГЭС___Венец_CN_207204995_220000_CN_121218185_220000/LConn2 -- Чебоксарская_ГЭС___Венец_CN_207204995_220000_CN_107692183_220000/LConn2 -- Чебоксарская_ГЭС___Венец_CN_207204995_220000_CN_93292147_220000/LConn2
  Чебоксарская_ГЭС___Венец_CN_207204995_220000_CN_305893253_220000/LConn3 -- T_207204995_220000;110000;6000_ПС_Венец_220_110_6_кВ/LConn3 -- Чебоксарская_ГЭС___Венец_CN_207204995_220000_CN_53366641_220000/LConn3 -- Чебоксарская_ГЭС___Венец_CN_207204995_220000_CN_121218185_220000/LConn3 -- Чебоксарская_ГЭС___Венец_CN_207204995_220000_CN_107692183_220000/LConn3 -- Чебоксарская_ГЭС___Венец_CN_207204995_220000_CN_93292147_220000/LConn3 -- bus188/LConn1
  T_305893253_220000;10000_ПС_Абашево_220_10_кВ/LConn1 -- Чебоксарская_ГЭС___Венец_CN_207204995_220000_CN_305893253_220000/RConn1
  T_305893253_220000;10000_ПС_Абашево_220_10_кВ/LConn2 -- Чебоксарская_ГЭС___Венец_CN_207204995_220000_CN_305893253_220000/RConn2
  Чебоксарская_ГЭС___Венец_CN_207204995_220000_CN_305893253_220000/RConn3 -- T_305893253_220000;10000_ПС_Абашево_220_10_кВ/LConn3 -- bus189/LConn1
  Чебоксарская_ГЭС___Венец_CN_207204995_220000_CN_53366641_220000/RConn1 -- T_53366641_220000;110000;6000_ПС_Канаш_220_110_6_кВ/LConn1 -- ВЛ_Канаш___Студенец_220_кВ_CN_274213600_220000_CN_53366641_220000/LConn1
  Чебоксарская_ГЭС___Венец_CN_207204995_220000_CN_53366641_220000/RConn2 -- T_53366641_220000;110000;6000_ПС_Канаш_220_110_6_кВ/LConn2 -- ВЛ_Канаш___Студенец_220_кВ_CN_274213600_220000_CN_53366641_220000/LConn2
  Чебоксарская_ГЭС___Венец_CN_207204995_220000_CN_53366641_220000/RConn3 -- T_53366641_220000;110000;6000_ПС_Канаш_220_110_6_кВ/LConn3 -- ВЛ_Канаш___Студенец_220_кВ_CN_274213600_220000_CN_53366641_220000/LConn3 -- bus190/LConn1
  T_121218185_220000;110000;10000_ПС_220_110_10_кВ_Тюрлема/LConn1 -- Чебоксарская_ГЭС___Венец_CN_207204995_220000_CN_121218185_220000/RConn1
  T_121218185_220000;110000;10000_ПС_220_110_10_кВ_Тюрлема/LConn2 -- Чебоксарская_ГЭС___Венец_CN_207204995_220000_CN_121218185_220000/RConn2
  Чебоксарская_ГЭС___Венец_CN_207204995_220000_CN_121218185_220000/RConn3 -- T_121218185_220000;110000;10000_ПС_220_110_10_кВ_Тюрлема/LConn3 -- bus191/LConn1
  Чебоксарская_ГЭС___Венец_CN_207204995_220000_CN_107692183_220000/RConn1 -- T_107692183_220000_ПС_Чигашево_220_110кВ/LConn1 -- Чигашево___Дубники_CN_224208787_220000_CN_107692183_220000/LConn1
  Чебоксарская_ГЭС___Венец_CN_207204995_220000_CN_107692183_220000/RConn2 -- T_107692183_220000_ПС_Чигашево_220_110кВ/LConn2 -- Чигашево___Дубники_CN_224208787_220000_CN_107692183_220000/LConn2
  Чебоксарская_ГЭС___Венец_CN_207204995_220000_CN_107692183_220000/RConn3 -- T_107692183_220000_ПС_Чигашево_220_110кВ/LConn3 -- Чигашево___Дубники_CN_224208787_220000_CN_107692183_220000/LConn3 -- bus192/LConn1
  Чебоксарская_ГЭС___Венец_CN_207204995_220000_CN_93292147_220000/RConn1 -- T_93292147_500000_ПС_Помары/RConn1 -- _CN_132783542_220000_CN_93292147_220000/LConn1 -- L_93292147/LConn1 -- _CN_137376045_220000_CN_93292147_220000/LConn1
  Чебоксарская_ГЭС___Венец_CN_207204995_220000_CN_93292147_220000/RConn2 -- T_93292147_500000_ПС_Помары/RConn2 -- _CN_132783542_220000_CN_93292147_220000/LConn2 -- L_93292147/LConn2 -- _CN_137376045_220000_CN_93292147_220000/LConn2
  Чебоксарская_ГЭС___Венец_CN_207204995_220000_CN_93292147_220000/RConn3 -- T_93292147_500000_ПС_Помары/RConn3 -- _CN_132783542_220000_CN_93292147_220000/LConn3 -- L_93292147/LConn3 -- bus193/LConn1 -- _CN_137376045_220000_CN_93292147_220000/LConn3
  T_305832836_220000_Лукояновская/LConn1 -- Арзамасская___Лукояновская_№1_CN_305832836_220000_CN_72288676_220000/RConn1
  T_305832836_220000_Лукояновская/LConn2 -- Арзамасская___Лукояновская_№1_CN_305832836_220000_CN_72288676_220000/RConn2
  Арзамасская___Лукояновская_№1_CN_305832836_220000_CN_72288676_220000/RConn3 -- T_305832836_220000_Лукояновская/LConn3 -- bus194/LConn1
  T_232164616__/LConn1 -- _CN_232164616_220000_CN_229942593_220000/LConn1
  T_232164616__/LConn2 -- _CN_232164616_220000_CN_229942593_220000/LConn2
  _CN_232164616_220000_CN_229942593_220000/LConn3 -- T_232164616__/LConn3 -- bus195/LConn1
  T_229942593__/LConn1 -- _CN_232164616_220000_CN_229942593_220000/RConn1
  T_229942593__/LConn2 -- _CN_232164616_220000_CN_229942593_220000/RConn2
  _CN_232164616_220000_CN_229942593_220000/RConn3 -- T_229942593__/LConn3 -- bus196/LConn1
  T_274937610_220000_ПС_220_кВ_Головная/LConn1 -- _CN_274937610_220000_CN_161082145_220000/LConn1
  T_274937610_220000_ПС_220_кВ_Головная/LConn2 -- _CN_274937610_220000_CN_161082145_220000/LConn2
  _CN_274937610_220000_CN_161082145_220000/LConn3 -- T_274937610_220000_ПС_220_кВ_Головная/LConn3 -- bus197/LConn1
  T_161082145_220000_ПС_220_кВ_Томыловская/LConn1 -- _CN_274937610_220000_CN_161082145_220000/RConn1
  T_161082145_220000_ПС_220_кВ_Томыловская/LConn2 -- _CN_274937610_220000_CN_161082145_220000/RConn2
  _CN_274937610_220000_CN_161082145_220000/RConn3 -- T_161082145_220000_ПС_220_кВ_Томыловская/LConn3 -- bus198/LConn1
  _CN_93494543_220000_CN_93508340_220000/LConn1 -- T_93494543_220000_Сеченово_1/LConn1 -- _CN_93494543_220000_CN_93494546_220000/LConn1
  _CN_93494543_220000_CN_93508340_220000/LConn2 -- T_93494543_220000_Сеченово_1/LConn2 -- _CN_93494543_220000_CN_93494546_220000/LConn2
  _CN_93494543_220000_CN_93508340_220000/LConn3 -- T_93494543_220000_Сеченово_1/LConn3 -- _CN_93494543_220000_CN_93494546_220000/LConn3 -- bus199/LConn1
  _CN_93494543_220000_CN_93508340_220000/RConn1 -- T_93508340_220000_Сеченово_2/LConn1 -- _CN_93494546_220000_CN_93508340_220000/LConn1
  _CN_93494543_220000_CN_93508340_220000/RConn2 -- T_93508340_220000_Сеченово_2/LConn2 -- _CN_93494546_220000_CN_93508340_220000/LConn2
  _CN_93494543_220000_CN_93508340_220000/RConn3 -- T_93508340_220000_Сеченово_2/LConn3 -- _CN_93494546_220000_CN_93508340_220000/LConn3 -- bus200/LConn1
  _CN_93494543_220000_CN_93494546_220000/RConn1 -- T_93494546_220000_РП_Сеченово/LConn1 -- Осиновка_РП_Сеченово_№2_CN_93494546_220000_CN_92419131_220000/LConn1 -- Сергач_РП_Сеченово_CN_93494546_220000_CN_277905350_220000/LConn1 -- _CN_93494546_220000_CN_93508340_220000/RConn1 -- Сеченово_Пильна_№2_CN_93494546_220000_CN_327138157_220000/LConn1
  _CN_93494543_220000_CN_93494546_220000/RConn2 -- T_93494546_220000_РП_Сеченово/LConn2 -- Осиновка_РП_Сеченово_№2_CN_93494546_220000_CN_92419131_220000/LConn2 -- Сергач_РП_Сеченово_CN_93494546_220000_CN_277905350_220000/LConn2 -- _CN_93494546_220000_CN_93508340_220000/RConn2 -- Сеченово_Пильна_№2_CN_93494546_220000_CN_327138157_220000/LConn2
  _CN_93494543_220000_CN_93494546_220000/RConn3 -- T_93494546_220000_РП_Сеченово/LConn3 -- Осиновка_РП_Сеченово_№2_CN_93494546_220000_CN_92419131_220000/LConn3 -- Сергач_РП_Сеченово_CN_93494546_220000_CN_277905350_220000/LConn3 -- bus201/LConn1 -- _CN_93494546_220000_CN_93508340_220000/RConn3 -- Сеченово_Пильна_№2_CN_93494546_220000_CN_327138157_220000/LConn3
  _CN_89430545_220000_CN_62194541_220000/LConn1 -- T_89430545__ПС_Киндери/RConn1 -- L_89430545/LConn1
  _CN_89430545_220000_CN_62194541_220000/LConn2 -- T_89430545__ПС_Киндери/RConn2 -- L_89430545/LConn2
  _CN_89430545_220000_CN_62194541_220000/LConn3 -- T_89430545__ПС_Киндери/RConn3 -- L_89430545/LConn3 -- bus202/LConn1
  T_62194541_220000_ПС_Магистральная/LConn1 -- _CN_89430545_220000_CN_62194541_220000/RConn1
  T_62194541_220000_ПС_Магистральная/LConn2 -- _CN_89430545_220000_CN_62194541_220000/RConn2
  _CN_89430545_220000_CN_62194541_220000/RConn3 -- T_62194541_220000_ПС_Магистральная/LConn3 -- bus203/LConn1
  "T_327138157_220000_ПС_220кВ_\"Пильна\""/LConn1 -- Сеченово_Пильна_№2_CN_93494546_220000_CN_327138157_220000/RConn1
  "T_327138157_220000_ПС_220кВ_\"Пильна\""/LConn2 -- Сеченово_Пильна_№2_CN_93494546_220000_CN_327138157_220000/RConn2
  Сеченово_Пильна_№2_CN_93494546_220000_CN_327138157_220000/RConn3 -- "T_327138157_220000_ПС_220кВ_\"Пильна\""/LConn3 -- bus204/LConn1
  Осиновка_РП_Сеченово_№2_CN_93494546_220000_CN_92419131_220000/RConn1 -- T_92419131_500000_Осиновка/RConn1 -- Рузаевка___Центролит_CN_113585698_220000_CN_92419131_220000/RConn1 -- Осиновка___Починковская_2_CN_92419131_220000_CN_327226015_220000/LConn1 -- Осиновка___Починковская_1_№2_CN_92419131_220000_CN_327226025_220000/LConn1 -- L_92419131/LConn1
  Осиновка_РП_Сеченово_№2_CN_93494546_220000_CN_92419131_220000/RConn2 -- T_92419131_500000_Осиновка/RConn2 -- Рузаевка___Центролит_CN_113585698_220000_CN_92419131_220000/RConn2 -- Осиновка___Починковская_2_CN_92419131_220000_CN_327226015_220000/LConn2 -- Осиновка___Починковская_1_№2_CN_92419131_220000_CN_327226025_220000/LConn2 -- L_92419131/LConn2
  Осиновка_РП_Сеченово_№2_CN_93494546_220000_CN_92419131_220000/RConn3 -- T_92419131_500000_Осиновка/RConn3 -- Рузаевка___Центролит_CN_113585698_220000_CN_92419131_220000/RConn3 -- Осиновка___Починковская_2_CN_92419131_220000_CN_327226015_220000/LConn3 -- Осиновка___Починковская_1_№2_CN_92419131_220000_CN_327226025_220000/LConn3 -- L_92419131/LConn3 -- bus205/LConn1
  Сергач_РП_Сеченово_CN_93494546_220000_CN_277905350_220000/RConn1 -- T_277905350_220000;110000_Сергач/LConn1 -- Арзамасская_Сергач_CN_72288676_220000_CN_277905350_220000/RConn1
  Сергач_РП_Сеченово_CN_93494546_220000_CN_277905350_220000/RConn2 -- T_277905350_220000;110000_Сергач/LConn2 -- Арзамасская_Сергач_CN_72288676_220000_CN_277905350_220000/RConn2
  Сергач_РП_Сеченово_CN_93494546_220000_CN_277905350_220000/RConn3 -- T_277905350_220000;110000_Сергач/LConn3 -- Арзамасская_Сергач_CN_72288676_220000_CN_277905350_220000/RConn3 -- bus206/LConn1
  T_224208787_220000_ПС_Дубники/LConn1 -- Чигашево___Дубники_CN_224208787_220000_CN_107692183_220000/RConn1
  T_224208787_220000_ПС_Дубники/LConn2 -- Чигашево___Дубники_CN_224208787_220000_CN_107692183_220000/RConn2
  Чигашево___Дубники_CN_224208787_220000_CN_107692183_220000/RConn3 -- T_224208787_220000_ПС_Дубники/LConn3 -- bus207/LConn1
  _CN_327325460_220000_CN_72288676_220000/RConn1 -- T_327325460_220000_Кудьма/LConn1 -- _CN_327325460_220000_CN_121048356_220000/LConn1
  _CN_327325460_220000_CN_72288676_220000/RConn2 -- T_327325460_220000_Кудьма/LConn2 -- _CN_327325460_220000_CN_121048356_220000/LConn2
  _CN_327325460_220000_CN_72288676_220000/RConn3 -- T_327325460_220000_Кудьма/LConn3 -- _CN_327325460_220000_CN_121048356_220000/LConn3 -- bus208/LConn1
  "T_121048356_220000_ПС_220кВ_\"Бобыльская\""/LConn1 -- _CN_327325460_220000_CN_121048356_220000/RConn1
  "T_121048356_220000_ПС_220кВ_\"Бобыльская\""/LConn2 -- _CN_327325460_220000_CN_121048356_220000/RConn2
  _CN_327325460_220000_CN_121048356_220000/RConn3 -- "T_121048356_220000_ПС_220кВ_\"Бобыльская\""/LConn3 -- bus209/LConn1
  T_171147802__/LConn1 -- _CN_171147802_220000_CN_240018999_220000/LConn1
  T_171147802__/LConn2 -- _CN_171147802_220000_CN_240018999_220000/LConn2
  _CN_171147802_220000_CN_240018999_220000/LConn3 -- T_171147802__/LConn3 -- bus210/LConn1
  T_240018999__/LConn1 -- _CN_171147802_220000_CN_240018999_220000/RConn1
  T_240018999__/LConn2 -- _CN_171147802_220000_CN_240018999_220000/RConn2
  _CN_171147802_220000_CN_240018999_220000/RConn3 -- T_240018999__/LConn3 -- bus211/LConn1
  T_158349339_220000_Подстанция_220_кВ_Космос/LConn1 -- _CN_158349339_220000_CN_128036424_220000/LConn1
  T_158349339_220000_Подстанция_220_кВ_Космос/LConn2 -- _CN_158349339_220000_CN_128036424_220000/LConn2
  _CN_158349339_220000_CN_128036424_220000/LConn3 -- T_158349339_220000_Подстанция_220_кВ_Космос/LConn3 -- bus212/LConn1
  _CN_158349339_220000_CN_128036424_220000/RConn1 -- T_128036424_500000;220000_Северная/RConn1 -- L_128036424/LConn1
  _CN_158349339_220000_CN_128036424_220000/RConn2 -- T_128036424_500000;220000_Северная/RConn2 -- L_128036424/LConn2
  _CN_158349339_220000_CN_128036424_220000/RConn3 -- T_128036424_500000;220000_Северная/RConn3 -- L_128036424/LConn3 -- bus213/LConn1
  _CN_306106528_220000_CN_328463572_220000/LConn1 -- T_306106528__Екатериновка_газовая/LConn1 -- _CN_306106528_220000_CN_224261932_220000/LConn1
  _CN_306106528_220000_CN_328463572_220000/LConn2 -- T_306106528__Екатериновка_газовая/LConn2 -- _CN_306106528_220000_CN_224261932_220000/LConn2
  _CN_306106528_220000_CN_328463572_220000/LConn3 -- T_306106528__Екатериновка_газовая/LConn3 -- _CN_306106528_220000_CN_224261932_220000/LConn3 -- bus214/LConn1
  T_328463572__/LConn1 -- _CN_306106528_220000_CN_328463572_220000/RConn1
  T_328463572__/LConn2 -- _CN_306106528_220000_CN_328463572_220000/RConn2
  _CN_306106528_220000_CN_328463572_220000/RConn3 -- T_328463572__/LConn3 -- bus215/LConn1
  T_224261932__Аткарская/LConn1 -- _CN_306106528_220000_CN_224261932_220000/RConn1
  T_224261932__Аткарская/LConn2 -- _CN_306106528_220000_CN_224261932_220000/RConn2
  _CN_306106528_220000_CN_224261932_220000/RConn3 -- T_224261932__Аткарская/LConn3 -- bus216/LConn1
  Рузаевка___Центролит_CN_113585698_220000_CN_327226015_220000/RConn1 -- T_327226015_220000_Починковская_2/LConn1 -- Осиновка___Починковская_2_CN_92419131_220000_CN_327226015_220000/RConn1
  Рузаевка___Центролит_CN_113585698_220000_CN_327226015_220000/RConn2 -- T_327226015_220000_Починковская_2/LConn2 -- Осиновка___Починковская_2_CN_92419131_220000_CN_327226015_220000/RConn2
  Рузаевка___Центролит_CN_113585698_220000_CN_327226015_220000/RConn3 -- T_327226015_220000_Починковская_2/LConn3 -- Осиновка___Починковская_2_CN_92419131_220000_CN_327226015_220000/RConn3 -- bus217/LConn1
  Рузаевка___Центролит_CN_113585698_220000_CN_103735794_220000/RConn1 -- T_103735794_220000_Центролит/LConn1 -- Центролит___Комсомольская_CN_276080500_220000_CN_103735794_220000/LConn1
  Рузаевка___Центролит_CN_113585698_220000_CN_103735794_220000/RConn2 -- T_103735794_220000_Центролит/LConn2 -- Центролит___Комсомольская_CN_276080500_220000_CN_103735794_220000/LConn2
  Рузаевка___Центролит_CN_113585698_220000_CN_103735794_220000/RConn3 -- T_103735794_220000_Центролит/LConn3 -- Центролит___Комсомольская_CN_276080500_220000_CN_103735794_220000/LConn3 -- bus218/LConn1
  T_48949159_220000;35000_/LConn1 -- _CN_48949159_220000_CN_51711046_220000/LConn1
  T_48949159_220000;35000_/LConn2 -- _CN_48949159_220000_CN_51711046_220000/LConn2
  _CN_48949159_220000_CN_51711046_220000/LConn3 -- T_48949159_220000;35000_/LConn3 -- bus219/LConn1
  T_51711046_220000;110000;fixme_/LConn1 -- _CN_48949159_220000_CN_51711046_220000/RConn1
  T_51711046_220000;110000;fixme_/LConn2 -- _CN_48949159_220000_CN_51711046_220000/RConn2
  _CN_48949159_220000_CN_51711046_220000/RConn3 -- T_51711046_220000;110000;fixme_/LConn3 -- bus220/LConn1
  T_276080500_220000_Комсомольская/LConn1 -- Центролит___Комсомольская_CN_276080500_220000_CN_103735794_220000/RConn1
  T_276080500_220000_Комсомольская/LConn2 -- Центролит___Комсомольская_CN_276080500_220000_CN_103735794_220000/RConn2
  Центролит___Комсомольская_CN_276080500_220000_CN_103735794_220000/RConn3 -- T_276080500_220000_Комсомольская/LConn3 -- bus221/LConn1
  T_96826924_220000;110000;10000_ПС_220_кВ_Новотроицкая/LConn1 -- _CN_96826924_220000_CN_97145033_220000/LConn1
  T_96826924_220000;110000;10000_ПС_220_кВ_Новотроицкая/LConn2 -- _CN_96826924_220000_CN_97145033_220000/LConn2
  _CN_96826924_220000_CN_97145033_220000/LConn3 -- T_96826924_220000;110000;10000_ПС_220_кВ_Новотроицкая/LConn3 -- bus222/LConn1
  T_97145033_220000;110000;10000_ПС_220_кВ_Орская/LConn1 -- _CN_96826924_220000_CN_97145033_220000/RConn1
  T_97145033_220000;110000;10000_ПС_220_кВ_Орская/LConn2 -- _CN_96826924_220000_CN_97145033_220000/RConn2
  _CN_96826924_220000_CN_97145033_220000/RConn3 -- T_97145033_220000;110000;10000_ПС_220_кВ_Орская/LConn3 -- bus223/LConn1
  T_137376045__/LConn1 -- _CN_137376045_220000_CN_93292147_220000/RConn1
  T_137376045__/LConn2 -- _CN_137376045_220000_CN_93292147_220000/RConn2
  _CN_137376045_220000_CN_93292147_220000/RConn3 -- T_137376045__/LConn3 -- bus224/LConn1
  T_132783542_220000_ПС_Волжская/LConn1 -- _CN_132783542_220000_CN_93292147_220000/RConn1
  T_132783542_220000_ПС_Волжская/LConn2 -- _CN_132783542_220000_CN_93292147_220000/RConn2
  _CN_132783542_220000_CN_93292147_220000/RConn3 -- T_132783542_220000_ПС_Волжская/LConn3 -- bus225/LConn1
  T_327226025_220000_Починковская_1/LConn1 -- Осиновка___Починковская_1_№2_CN_92419131_220000_CN_327226025_220000/RConn1
  T_327226025_220000_Починковская_1/LConn2 -- Осиновка___Починковская_1_№2_CN_92419131_220000_CN_327226025_220000/RConn2
  Осиновка___Починковская_1_№2_CN_92419131_220000_CN_327226025_220000/RConn3 -- T_327226025_220000_Починковская_1/LConn3 -- bus226/LConn1
  T_94214974__ПС_Нижнекамская/LConn1 -- _CN_94214974_220000_CN_104227388_220000/LConn1
  T_94214974__ПС_Нижнекамская/LConn2 -- _CN_94214974_220000_CN_104227388_220000/LConn2
  _CN_94214974_220000_CN_104227388_220000/LConn3 -- T_94214974__ПС_Нижнекамская/LConn3 -- bus227/LConn1
  G_104227388_НкТЭЦ_2/RConn1 -- _CN_94214974_220000_CN_104227388_220000/RConn1
  G_104227388_НкТЭЦ_2/RConn2 -- _CN_94214974_220000_CN_104227388_220000/RConn2
  _CN_94214974_220000_CN_104227388_220000/RConn3 -- G_104227388_НкТЭЦ_2/RConn3 -- bus228/LConn1
  T_96563667__/LConn1 -- _CN_96563667_220000_CN_83478009_220000/LConn1
  T_96563667__/LConn2 -- _CN_96563667_220000_CN_83478009_220000/LConn2
  _CN_96563667_220000_CN_83478009_220000/LConn3 -- T_96563667__/LConn3 -- bus229/LConn1
  _CN_96563667_220000_CN_83478009_220000/RConn1 -- G_83478009_Пермская_ГРЭС/RConn1 -- _CN_193513250_500000_CN_83478009_220000/LConn1
  _CN_96563667_220000_CN_83478009_220000/RConn2 -- G_83478009_Пермская_ГРЭС/RConn2 -- _CN_193513250_500000_CN_83478009_220000/LConn2
  _CN_96563667_220000_CN_83478009_220000/RConn3 -- G_83478009_Пермская_ГРЭС/RConn3 -- _CN_193513250_500000_CN_83478009_220000/LConn3 -- bus230/LConn1
  T_95488527_220000;110000;35000;6000_ПС_Абдрахманово/LConn1 -- _CN_95488527_220000_CN_95488500_220000/LConn1
  T_95488527_220000;110000;35000;6000_ПС_Абдрахманово/LConn2 -- _CN_95488527_220000_CN_95488500_220000/LConn2
  _CN_95488527_220000_CN_95488500_220000/LConn3 -- T_95488527_220000;110000;35000;6000_ПС_Абдрахманово/LConn3 -- bus231/LConn1
  T_95488500__ПС_Письмянка/LConn1 -- _CN_95488527_220000_CN_95488500_220000/RConn1
  T_95488500__ПС_Письмянка/LConn2 -- _CN_95488527_220000_CN_95488500_220000/RConn2
  _CN_95488527_220000_CN_95488500_220000/RConn3 -- T_95488500__ПС_Письмянка/LConn3 -- bus232/LConn1
  T_274213600_220000_ПС_Студенец/LConn1 -- ВЛ_Канаш___Студенец_220_кВ_CN_274213600_220000_CN_53366641_220000/RConn1
  T_274213600_220000_ПС_Студенец/LConn2 -- ВЛ_Канаш___Студенец_220_кВ_CN_274213600_220000_CN_53366641_220000/RConn2
  ВЛ_Канаш___Студенец_220_кВ_CN_274213600_220000_CN_53366641_220000/RConn3 -- T_274213600_220000_ПС_Студенец/LConn3 -- bus233/LConn1
  T_82458858_220000_ОРУ_220_кВ/LConn1 -- _CN_82458858_220000_CN_273327356_110000/RConn1
  T_82458858_220000_ОРУ_220_кВ/LConn2 -- _CN_82458858_220000_CN_273327356_110000/RConn2
  _CN_82458858_220000_CN_273327356_110000/RConn3 -- T_82458858_220000_ОРУ_220_кВ/LConn3 -- bus234/LConn1
  _CN_110601218_500000_CN_245072101_110000/RConn1 -- T_110601218_500000_/LConn1 -- _CN_110601218_500000_CN_131490223_500000/LConn1 -- _CN_110601218_500000_CN_136586702_500000/LConn1
  _CN_110601218_500000_CN_245072101_110000/RConn2 -- T_110601218_500000_/LConn2 -- _CN_110601218_500000_CN_131490223_500000/LConn2 -- _CN_110601218_500000_CN_136586702_500000/LConn2
  _CN_110601218_500000_CN_245072101_110000/RConn3 -- T_110601218_500000_/LConn3 -- _CN_110601218_500000_CN_131490223_500000/LConn3 -- _CN_110601218_500000_CN_136586702_500000/LConn3 -- bus235/LConn1
  _CN_110601218_500000_CN_131490223_500000/RConn1 -- T_131490223__ПС_Вешкайма/LConn1 -- Вешкайма_Арзамасская_CN_72288676_500000_CN_131490223_500000/LConn1 -- ВЛ_Вешкайма_Пенза_2_500кВ_CN_131490223_500000_CN_82967790_500000/LConn1 -- _CN_131490223_500000_CN_92419131_500000/LConn1 -- ВЛ_Вешкайма_Ключики_500кВ_CN_131508245_500000_CN_131490223_500000/LConn1
  _CN_110601218_500000_CN_131490223_500000/RConn2 -- T_131490223__ПС_Вешкайма/LConn2 -- Вешкайма_Арзамасская_CN_72288676_500000_CN_131490223_500000/LConn2 -- ВЛ_Вешкайма_Пенза_2_500кВ_CN_131490223_500000_CN_82967790_500000/LConn2 -- _CN_131490223_500000_CN_92419131_500000/LConn2 -- ВЛ_Вешкайма_Ключики_500кВ_CN_131508245_500000_CN_131490223_500000/LConn2
  _CN_110601218_500000_CN_131490223_500000/RConn3 -- T_131490223__ПС_Вешкайма/LConn3 -- Вешкайма_Арзамасская_CN_72288676_500000_CN_131490223_500000/LConn3 -- ВЛ_Вешкайма_Пенза_2_500кВ_CN_131490223_500000_CN_82967790_500000/LConn3 -- _CN_131490223_500000_CN_92419131_500000/LConn3 -- bus236/LConn1 -- ВЛ_Вешкайма_Ключики_500кВ_CN_131508245_500000_CN_131490223_500000/LConn3
  _CN_110601218_500000_CN_136586702_500000/RConn1 -- T_136586702_500000;220000;110000_ПС_Азот/LConn1 -- ВЛ_Азот___Бугульма_500кВ_CN_88028486_500000_CN_136586702_500000/LConn1
  _CN_110601218_500000_CN_136586702_500000/RConn2 -- T_136586702_500000;220000;110000_ПС_Азот/LConn2 -- ВЛ_Азот___Бугульма_500кВ_CN_88028486_500000_CN_136586702_500000/LConn2
  _CN_110601218_500000_CN_136586702_500000/RConn3 -- T_136586702_500000;220000;110000_ПС_Азот/LConn3 -- ВЛ_Азот___Бугульма_500кВ_CN_88028486_500000_CN_136586702_500000/LConn3 -- bus237/LConn1
  ВЛ_500кВ_Буйская___Калино_CN_219655813_500000_CN_53015400_500000/LConn1 -- T_219655813_500000;220000;110000_ПС_Буйская/LConn1 -- ВЛ_500кВ_КарГРЭС___Буйская_CN_219655813_500000_CN_376942192_500000/LConn1 -- ВЛ_500кВ_Буйская___Уфимская_CN_219655813_500000_CN_114285735_500000/LConn1
  ВЛ_500кВ_Буйская___Калино_CN_219655813_500000_CN_53015400_500000/LConn2 -- T_219655813_500000;220000;110000_ПС_Буйская/LConn2 -- ВЛ_500кВ_КарГРЭС___Буйская_CN_219655813_500000_CN_376942192_500000/LConn2 -- ВЛ_500кВ_Буйская___Уфимская_CN_219655813_500000_CN_114285735_500000/LConn2
  ВЛ_500кВ_Буйская___Калино_CN_219655813_500000_CN_53015400_500000/LConn3 -- T_219655813_500000;220000;110000_ПС_Буйская/LConn3 -- ВЛ_500кВ_КарГРЭС___Буйская_CN_219655813_500000_CN_376942192_500000/LConn3 -- ВЛ_500кВ_Буйская___Уфимская_CN_219655813_500000_CN_114285735_500000/LConn3 -- bus238/LConn1
  ВЛ_500кВ_Буйская___Калино_CN_219655813_500000_CN_53015400_500000/RConn1 -- T_53015400_500000_ПС_Калино/LConn1 -- _CN_193513250_500000_CN_53015400_500000/LConn1
  ВЛ_500кВ_Буйская___Калино_CN_219655813_500000_CN_53015400_500000/RConn2 -- T_53015400_500000_ПС_Калино/LConn2 -- _CN_193513250_500000_CN_53015400_500000/LConn2
  ВЛ_500кВ_Буйская___Калино_CN_219655813_500000_CN_53015400_500000/RConn3 -- T_53015400_500000_ПС_Калино/LConn3 -- _CN_193513250_500000_CN_53015400_500000/LConn3 -- bus239/LConn1
  ВЛ_500кВ_КарГРЭС___Буйская_CN_219655813_500000_CN_376942192_500000/RConn1 -- T_376942192__/LConn1 -- ВЛ_КарГРЭС_Удмуртская_500кВ_CN_229649869_500000_CN_376942192_500000/LConn1
  ВЛ_500кВ_КарГРЭС___Буйская_CN_219655813_500000_CN_376942192_500000/RConn2 -- T_376942192__/LConn2 -- ВЛ_КарГРЭС_Удмуртская_500кВ_CN_229649869_500000_CN_376942192_500000/LConn2
  ВЛ_500кВ_КарГРЭС___Буйская_CN_219655813_500000_CN_376942192_500000/RConn3 -- T_376942192__/LConn3 -- ВЛ_КарГРЭС_Удмуртская_500кВ_CN_229649869_500000_CN_376942192_500000/LConn3 -- bus240/LConn1
  T_114285735_500000;220000;10000_ПС_Уфимская/LConn1 -- ВЛ_500кВ_Буйская___Уфимская_CN_219655813_500000_CN_114285735_500000/RConn1
  T_114285735_500000;220000;10000_ПС_Уфимская/LConn2 -- ВЛ_500кВ_Буйская___Уфимская_CN_219655813_500000_CN_114285735_500000/RConn2
  ВЛ_500кВ_Буйская___Уфимская_CN_219655813_500000_CN_114285735_500000/RConn3 -- T_114285735_500000;220000;10000_ПС_Уфимская/LConn3 -- bus241/LConn1
  T_92325642_500000_Радуга/LConn1 -- Арзамасская___Радуга_Северная_CN_92325642_500000_CN_72288676_500000/LConn1
  T_92325642_500000_Радуга/LConn2 -- Арзамасская___Радуга_Северная_CN_92325642_500000_CN_72288676_500000/LConn2
  Арзамасская___Радуга_Северная_CN_92325642_500000_CN_72288676_500000/LConn3 -- T_92325642_500000_Радуга/LConn3 -- bus242/LConn1
  Арзамасская___Радуга_Северная_CN_92325642_500000_CN_72288676_500000/RConn1 -- T_72288676_500000_Арзамасская/LConn1 -- Вешкайма_Арзамасская_CN_72288676_500000_CN_131490223_500000/RConn1 -- Арзамасская_Осиновка_CN_72288676_500000_CN_92419131_500000/LConn1
  Арзамасская___Радуга_Северная_CN_92325642_500000_CN_72288676_500000/RConn2 -- T_72288676_500000_Арзамасская/LConn2 -- Вешкайма_Арзамасская_CN_72288676_500000_CN_131490223_500000/RConn2 -- Арзамасская_Осиновка_CN_72288676_500000_CN_92419131_500000/LConn2
  Арзамасская___Радуга_Северная_CN_92325642_500000_CN_72288676_500000/RConn3 -- T_72288676_500000_Арзамасская/LConn3 -- Вешкайма_Арзамасская_CN_72288676_500000_CN_131490223_500000/RConn3 -- Арзамасская_Осиновка_CN_72288676_500000_CN_92419131_500000/LConn3 -- bus243/LConn1
  ВЛ_500кВ_Бугульма___Бекетово_CN_150285837_500000_CN_88028486_500000/LConn1 -- T_150285837_500000;220000;110000_ПС_Бекетово/LConn1 -- ВЛ_500кВ_Смеловская_Бекетово_CN_150285837_500000_CN_99190583_500000/LConn1
  ВЛ_500кВ_Бугульма___Бекетово_CN_150285837_500000_CN_88028486_500000/LConn2 -- T_150285837_500000;220000;110000_ПС_Бекетово/LConn2 -- ВЛ_500кВ_Смеловская_Бекетово_CN_150285837_500000_CN_99190583_500000/LConn2
  ВЛ_500кВ_Бугульма___Бекетово_CN_150285837_500000_CN_88028486_500000/LConn3 -- T_150285837_500000;220000;110000_ПС_Бекетово/LConn3 -- ВЛ_500кВ_Смеловская_Бекетово_CN_150285837_500000_CN_99190583_500000/LConn3 -- bus244/LConn1
  ВЛ_500кВ_Бугульма___Бекетово_CN_150285837_500000_CN_88028486_500000/RConn1 -- "T_88028486_500000_ПС_500_кВ_\"Бугульма\""/LConn1 -- ВЛ_Азот___Бугульма_500кВ_CN_88028486_500000_CN_136586702_500000/RConn1
  ВЛ_500кВ_Бугульма___Бекетово_CN_150285837_500000_CN_88028486_500000/RConn2 -- "T_88028486_500000_ПС_500_кВ_\"Бугульма\""/LConn2 -- ВЛ_Азот___Бугульма_500кВ_CN_88028486_500000_CN_136586702_500000/RConn2
  ВЛ_500кВ_Бугульма___Бекетово_CN_150285837_500000_CN_88028486_500000/RConn3 -- "T_88028486_500000_ПС_500_кВ_\"Бугульма\""/LConn3 -- ВЛ_Азот___Бугульма_500кВ_CN_88028486_500000_CN_136586702_500000/RConn3 -- bus245/LConn1
  ВЛ_500кВ_Смеловская_Бекетово_CN_150285837_500000_CN_99190583_500000/RConn1 -- "T_99190583_500000;220000;110000;fixme_\"Смеловская\"_500_кВ"/LConn1 -- _CN_219112646_500000_CN_99190583_500000/LConn1
  ВЛ_500кВ_Смеловская_Бекетово_CN_150285837_500000_CN_99190583_500000/RConn2 -- "T_99190583_500000;220000;110000;fixme_\"Смеловская\"_500_кВ"/LConn2 -- _CN_219112646_500000_CN_99190583_500000/LConn2
  ВЛ_500кВ_Смеловская_Бекетово_CN_150285837_500000_CN_99190583_500000/RConn3 -- "T_99190583_500000;220000;110000;fixme_\"Смеловская\"_500_кВ"/LConn3 -- _CN_219112646_500000_CN_99190583_500000/LConn3 -- bus246/LConn1
  T_89430545__ПС_Киндери/LConn1 -- ВЛ_Помары_Киндери_500кВ_CN_89430545_500000_CN_93292147_500000/LConn1
  T_89430545__ПС_Киндери/LConn2 -- ВЛ_Помары_Киндери_500кВ_CN_89430545_500000_CN_93292147_500000/LConn2
  ВЛ_Помары_Киндери_500кВ_CN_89430545_500000_CN_93292147_500000/LConn3 -- T_89430545__ПС_Киндери/LConn3 -- bus247/LConn1
  T_93292147_500000_ПС_Помары/LConn1 -- ВЛ_Помары_Киндери_500кВ_CN_89430545_500000_CN_93292147_500000/RConn1
  T_93292147_500000_ПС_Помары/LConn2 -- ВЛ_Помары_Киндери_500кВ_CN_89430545_500000_CN_93292147_500000/RConn2
  ВЛ_Помары_Киндери_500кВ_CN_89430545_500000_CN_93292147_500000/RConn3 -- T_93292147_500000_ПС_Помары/LConn3 -- bus248/LConn1
  T_131508245_500000_ПС_Ключики/LConn1 -- ВЛ_Вешкайма_Ключики_500кВ_CN_131508245_500000_CN_131490223_500000/RConn1
  T_131508245_500000_ПС_Ключики/LConn2 -- ВЛ_Вешкайма_Ключики_500кВ_CN_131508245_500000_CN_131490223_500000/RConn2
  ВЛ_Вешкайма_Ключики_500кВ_CN_131508245_500000_CN_131490223_500000/RConn3 -- T_131508245_500000_ПС_Ключики/LConn3 -- bus249/LConn1
  _CN_193513250_500000_CN_128036424_500000/LConn1 -- T_193513250__/LConn1 -- _CN_193513250_500000_CN_83478009_220000/RConn1 -- _CN_193513250_500000_CN_53015400_500000/RConn1
  _CN_193513250_500000_CN_128036424_500000/LConn2 -- T_193513250__/LConn2 -- _CN_193513250_500000_CN_83478009_220000/RConn2 -- _CN_193513250_500000_CN_53015400_500000/RConn2
  _CN_193513250_500000_CN_128036424_500000/LConn3 -- T_193513250__/LConn3 -- _CN_193513250_500000_CN_83478009_220000/RConn3 -- bus250/LConn1 -- _CN_193513250_500000_CN_53015400_500000/RConn3
  T_128036424_500000;220000_Северная/LConn1 -- _CN_193513250_500000_CN_128036424_500000/RConn1
  T_128036424_500000;220000_Северная/LConn2 -- _CN_193513250_500000_CN_128036424_500000/RConn2
  _CN_193513250_500000_CN_128036424_500000/RConn3 -- T_128036424_500000;220000_Северная/LConn3 -- bus251/LConn1
  Арзамасская_Осиновка_CN_72288676_500000_CN_92419131_500000/RConn1 -- T_92419131_500000_Осиновка/LConn1 -- _CN_131490223_500000_CN_92419131_500000/RConn1
  Арзамасская_Осиновка_CN_72288676_500000_CN_92419131_500000/RConn2 -- T_92419131_500000_Осиновка/LConn2 -- _CN_131490223_500000_CN_92419131_500000/RConn2
  Арзамасская_Осиновка_CN_72288676_500000_CN_92419131_500000/RConn3 -- T_92419131_500000_Осиновка/LConn3 -- _CN_131490223_500000_CN_92419131_500000/RConn3 -- bus252/LConn1
  _CN_219112646_500000_CN_363144177_500000/LConn1 -- T_219112646__/LConn1 -- _CN_219112646_500000_CN_99190583_500000/RConn1
  _CN_219112646_500000_CN_363144177_500000/LConn2 -- T_219112646__/LConn2 -- _CN_219112646_500000_CN_99190583_500000/RConn2
  _CN_219112646_500000_CN_363144177_500000/LConn3 -- T_219112646__/LConn3 -- _CN_219112646_500000_CN_99190583_500000/RConn3 -- bus253/LConn1
  T_363144177__ОРУ_500_кВ_ИрГРЭС___1/LConn1 -- _CN_219112646_500000_CN_363144177_500000/RConn1
  T_363144177__ОРУ_500_кВ_ИрГРЭС___1/LConn2 -- _CN_219112646_500000_CN_363144177_500000/RConn2
  _CN_219112646_500000_CN_363144177_500000/RConn3 -- T_363144177__ОРУ_500_кВ_ИрГРЭС___1/LConn3 -- bus254/LConn1
  T_90273320__Курдюм/LConn1 -- _CN_90273320_500000_CN_48906740_500000/LConn1
  T_90273320__Курдюм/LConn2 -- _CN_90273320_500000_CN_48906740_500000/LConn2
  _CN_90273320_500000_CN_48906740_500000/LConn3 -- T_90273320__Курдюм/LConn3 -- bus255/LConn1
  _CN_90273320_500000_CN_48906740_500000/RConn1 -- G_48906740_Балаковская_АЭС/RConn1 -- _CN_227835712_500000_CN_48906740_500000/LConn1
  _CN_90273320_500000_CN_48906740_500000/RConn2 -- G_48906740_Балаковская_АЭС/RConn2 -- _CN_227835712_500000_CN_48906740_500000/LConn2
  _CN_90273320_500000_CN_48906740_500000/RConn3 -- G_48906740_Балаковская_АЭС/RConn3 -- _CN_227835712_500000_CN_48906740_500000/LConn3 -- bus256/LConn1
  T_82967790__ПС_Пенза_2/LConn1 -- ВЛ_Вешкайма_Пенза_2_500кВ_CN_131490223_500000_CN_82967790_500000/RConn1
  T_82967790__ПС_Пенза_2/LConn2 -- ВЛ_Вешкайма_Пенза_2_500кВ_CN_131490223_500000_CN_82967790_500000/RConn2
  ВЛ_Вешкайма_Пенза_2_500кВ_CN_131490223_500000_CN_82967790_500000/RConn3 -- T_82967790__ПС_Пенза_2/LConn3 -- bus257/LConn1
  T_227835712_500000;220000_ПС_500_кВ_Красноармейская/LConn1 -- _CN_227835712_500000_CN_48906740_500000/RConn1
  T_227835712_500000;220000_ПС_500_кВ_Красноармейская/LConn2 -- _CN_227835712_500000_CN_48906740_500000/RConn2
  _CN_227835712_500000_CN_48906740_500000/RConn3 -- T_227835712_500000;220000_ПС_500_кВ_Красноармейская/LConn3 -- bus258/LConn1
  T_229649869_500000_ПС_500_кВ_Удмуртская/LConn1 -- ВЛ_КарГРЭС_Удмуртская_500кВ_CN_229649869_500000_CN_376942192_500000/RConn1
  T_229649869_500000_ПС_500_кВ_Удмуртская/LConn2 -- ВЛ_КарГРЭС_Удмуртская_500кВ_CN_229649869_500000_CN_376942192_500000/RConn2
  ВЛ_КарГРЭС_Удмуртская_500кВ_CN_229649869_500000_CN_376942192_500000/RConn3 -- T_229649869_500000_ПС_500_кВ_Удмуртская/LConn3 -- bus259/LConn1
  T_82459105_500000_ОРУ_500_кВ/LConn1 -- _CN_82459105_500000_CN_273327356_110000/RConn1
  T_82459105_500000_ОРУ_500_кВ/LConn2 -- _CN_82459105_500000_CN_273327356_110000/RConn2
  _CN_82459105_500000_CN_273327356_110000/RConn3 -- T_82459105_500000_ОРУ_500_кВ/LConn3 -- bus260/LConn1
  T_169556579__ПC_Приваловская_500_кВ/LConn1 -- ВЛ_500кВ_Кропачево___Приваловская_CN_169556579_500000_CN_113767652_500000/LConn1
  T_169556579__ПC_Приваловская_500_кВ/LConn2 -- ВЛ_500кВ_Кропачево___Приваловская_CN_169556579_500000_CN_113767652_500000/LConn2
  ВЛ_500кВ_Кропачево___Приваловская_CN_169556579_500000_CN_113767652_500000/LConn3 -- T_169556579__ПC_Приваловская_500_кВ/LConn3 -- bus261/LConn1
  T_113767652_500000_ПС_Кропачево/LConn1 -- ВЛ_500кВ_Кропачево___Приваловская_CN_169556579_500000_CN_113767652_500000/RConn1
  T_113767652_500000_ПС_Кропачево/LConn2 -- ВЛ_500кВ_Кропачево___Приваловская_CN_169556579_500000_CN_113767652_500000/RConn2
  ВЛ_500кВ_Кропачево___Приваловская_CN_169556579_500000_CN_113767652_500000/RConn3 -- T_113767652_500000_ПС_Кропачево/LConn3 -- bus262/LConn1
  T_218733056__/RConn1 -- L_218733056/LConn1
  T_218733056__/RConn2 -- L_218733056/LConn2
  L_218733056/LConn3 -- T_218733056__/RConn3 -- bus263/LConn1
  T_218733818__/RConn1 -- L_218733818/LConn1
  T_218733818__/RConn2 -- L_218733818/LConn2
  L_218733818/LConn3 -- T_218733818__/RConn3 -- bus264/LConn1
  T_218733820__/RConn1 -- L_218733820/LConn1
  T_218733820__/RConn2 -- L_218733820/LConn2
  L_218733820/LConn3 -- T_218733820__/RConn3 -- bus265/LConn1
  T_107942401__/RConn1 -- L_107942401/LConn1
  T_107942401__/RConn2 -- L_107942401/LConn2
  L_107942401/LConn3 -- T_107942401__/RConn3 -- bus266/LConn1
  T_90682372__/RConn1 -- L_90682372/LConn1
  T_90682372__/RConn2 -- L_90682372/LConn2
  L_90682372/LConn3 -- T_90682372__/RConn3 -- bus267/LConn1
  T_67498838__ПС_Заводская/RConn1 -- L_67498838/LConn1
  T_67498838__ПС_Заводская/RConn2 -- L_67498838/LConn2
  L_67498838/LConn3 -- T_67498838__ПС_Заводская/RConn3 -- bus268/LConn1
  T_329997654_110000_/RConn1 -- L_329997654/LConn1
  T_329997654_110000_/RConn2 -- L_329997654/LConn2
  L_329997654/LConn3 -- T_329997654_110000_/RConn3 -- bus269/LConn1
  T_283379848_220000_ПС_220_кВ_Сива/RConn1 -- L_283379848/LConn1
  T_283379848_220000_ПС_220_кВ_Сива/RConn2 -- L_283379848/LConn2
  L_283379848/LConn3 -- T_283379848_220000_ПС_220_кВ_Сива/RConn3 -- bus270/LConn1
  T_280247962_110000;10000_ПС_110_10_кВ_Нискасы/RConn1 -- L_280247962/LConn1
  T_280247962_110000;10000_ПС_110_10_кВ_Нискасы/RConn2 -- L_280247962/LConn2
  L_280247962/LConn3 -- T_280247962_110000;10000_ПС_110_10_кВ_Нискасы/RConn3 -- bus271/LConn1
  T_280247969_110000;35000;10000_ПС_110_35_10_кВ_Моргауши/RConn1 -- L_280247969/LConn1
  T_280247969_110000;35000;10000_ПС_110_35_10_кВ_Моргауши/RConn2 -- L_280247969/LConn2
  L_280247969/LConn3 -- T_280247969_110000;35000;10000_ПС_110_35_10_кВ_Моргауши/RConn3 -- bus272/LConn1
  T_160723975_110000;35000;10000_ПС_110_35_10_кВ_Чапаевская/RConn1 -- L_160723975/LConn1
  T_160723975_110000;35000;10000_ПС_110_35_10_кВ_Чапаевская/RConn2 -- L_160723975/LConn2
  L_160723975/LConn3 -- T_160723975_110000;35000;10000_ПС_110_35_10_кВ_Чапаевская/RConn3 -- bus273/LConn1
  T_165640869__/RConn1 -- L_165640869/LConn1
  T_165640869__/RConn2 -- L_165640869/LConn2
  L_165640869/LConn3 -- T_165640869__/RConn3 -- bus274/LConn1
  T_137714986__/RConn1 -- L_137714986/LConn1
  T_137714986__/RConn2 -- L_137714986/LConn2
  L_137714986/LConn3 -- T_137714986__/RConn3 -- bus275/LConn1
  T_227673096_110000;10000_ПС_110_10кВ_Алтышево/RConn1 -- L_227673096/LConn1
  T_227673096_110000;10000_ПС_110_10кВ_Алтышево/RConn2 -- L_227673096/LConn2
  L_227673096/LConn3 -- T_227673096_110000;10000_ПС_110_10кВ_Алтышево/RConn3 -- bus276/LConn1
  T_219889824_110000;35000;6000_ПС_110_35_6_кВ_Алатырь/RConn1 -- L_219889824/LConn1
  T_219889824_110000;35000;6000_ПС_110_35_6_кВ_Алатырь/RConn2 -- L_219889824/LConn2
  L_219889824/LConn3 -- T_219889824_110000;35000;6000_ПС_110_35_6_кВ_Алатырь/RConn3 -- bus277/LConn1
  T_279919302_110000;10000_ПС_110_10_кВ_Первомайская/RConn1 -- L_279919302/LConn1
  T_279919302_110000;10000_ПС_110_10_кВ_Первомайская/RConn2 -- L_279919302/LConn2
  L_279919302/LConn3 -- T_279919302_110000;10000_ПС_110_10_кВ_Первомайская/RConn3 -- bus278/LConn1
  T_279919300_110000;35000;10000_ПС_110_35_10_кВ_Шемурша/RConn1 -- L_279919300/LConn1
  T_279919300_110000;35000;10000_ПС_110_35_10_кВ_Шемурша/RConn2 -- L_279919300/LConn2
  L_279919300/LConn3 -- T_279919300_110000;35000;10000_ПС_110_35_10_кВ_Шемурша/RConn3 -- bus279/LConn1
  T_279978585_110000;10000_ПС_110_10_кВ_Буинск/RConn1 -- L_279978585/LConn1
  T_279978585_110000;10000_ПС_110_10_кВ_Буинск/RConn2 -- L_279978585/LConn2
  L_279978585/LConn3 -- T_279978585_110000;10000_ПС_110_10_кВ_Буинск/RConn3 -- bus280/LConn1
  T_279978586_110000;10000_ПС_110_10_кВ_Ибреси/RConn1 -- L_279978586/LConn1
  T_279978586_110000;10000_ПС_110_10_кВ_Ибреси/RConn2 -- L_279978586/LConn2
  L_279978586/LConn3 -- T_279978586_110000;10000_ПС_110_10_кВ_Ибреси/RConn3 -- bus281/LConn1
  T_279978587_110000;10000_ПС_110_10_кВ_Рассвет/RConn1 -- L_279978587/LConn1
  T_279978587_110000;10000_ПС_110_10_кВ_Рассвет/RConn2 -- L_279978587/LConn2
  L_279978587/LConn3 -- T_279978587_110000;10000_ПС_110_10_кВ_Рассвет/RConn3 -- bus282/LConn1
  T_242619649_110000;10000_ПС_110_10_кВ_Чагаси/RConn1 -- L_242619649/LConn1
  T_242619649_110000;10000_ПС_110_10_кВ_Чагаси/RConn2 -- L_242619649/LConn2
  L_242619649/LConn3 -- T_242619649_110000;10000_ПС_110_10_кВ_Чагаси/RConn3 -- bus283/LConn1
  T_198002186_110000;10000_ПС_110_10_кВ_Бройлерная/RConn1 -- L_198002186/LConn1
  T_198002186_110000;10000_ПС_110_10_кВ_Бройлерная/RConn2 -- L_198002186/LConn2
  L_198002186/LConn3 -- T_198002186_110000;10000_ПС_110_10_кВ_Бройлерная/RConn3 -- bus284/LConn1
  T_197887411_110000;35000;10000_ПС_110_35_10_кВ_Атлашево/RConn1 -- L_197887411/LConn1
  T_197887411_110000;35000;10000_ПС_110_35_10_кВ_Атлашево/RConn2 -- L_197887411/LConn2
  L_197887411/LConn3 -- T_197887411_110000;35000;10000_ПС_110_35_10_кВ_Атлашево/RConn3 -- bus285/LConn1
  T_311468947__ОРУ_ТЭЦ_3/RConn1 -- L_311468947/LConn1
  T_311468947__ОРУ_ТЭЦ_3/RConn2 -- L_311468947/LConn2
  L_311468947/LConn3 -- T_311468947__ОРУ_ТЭЦ_3/RConn3 -- bus286/LConn1
  T_234246987_110000;10000_ПС_110_10_кВ_Луч/RConn1 -- L_234246987/LConn1
  T_234246987_110000;10000_ПС_110_10_кВ_Луч/RConn2 -- L_234246987/LConn2
  L_234246987/LConn3 -- T_234246987_110000;10000_ПС_110_10_кВ_Луч/RConn3 -- bus287/LConn1
  T_281834842_110000;35000;10000_ПС_110_35_10_кВ_Катраси/RConn1 -- L_281834842/LConn1
  T_281834842_110000;35000;10000_ПС_110_35_10_кВ_Катраси/RConn2 -- L_281834842/LConn2
  L_281834842/LConn3 -- T_281834842_110000;35000;10000_ПС_110_35_10_кВ_Катраси/RConn3 -- bus288/LConn1
  T_180390411__ПС_Бугульма/RConn1 -- L_180390411/LConn1
  T_180390411__ПС_Бугульма/RConn2 -- L_180390411/LConn2
  L_180390411/LConn3 -- T_180390411__ПС_Бугульма/RConn3 -- bus289/LConn1
  T_238549570__ПС_Алкино/RConn1 -- L_238549570/LConn1
  T_238549570__ПС_Алкино/RConn2 -- L_238549570/LConn2
  L_238549570/LConn3 -- T_238549570__ПС_Алкино/RConn3 -- bus290/LConn1
  T_82459148_110000_ОРУ_110_кВ/RConn1 -- L_82459148/LConn1
  T_82459148_110000_ОРУ_110_кВ/RConn2 -- L_82459148/LConn2
  L_82459148/LConn3 -- T_82459148_110000_ОРУ_110_кВ/RConn3 -- bus291/LConn1
  T_104554513__/RConn1 -- L_104554513/LConn1
  T_104554513__/RConn2 -- L_104554513/LConn2
  L_104554513/LConn3 -- T_104554513__/RConn3 -- bus292/LConn1
  T_320965592__/RConn1 -- L_320965592/LConn1
  T_320965592__/RConn2 -- L_320965592/LConn2
  L_320965592/LConn3 -- T_320965592__/RConn3 -- bus293/LConn1
  T_93482528__/RConn1 -- L_93482528/LConn1
  T_93482528__/RConn2 -- L_93482528/LConn2
  L_93482528/LConn3 -- T_93482528__/RConn3 -- bus294/LConn1
  T_158349331__/RConn1 -- L_158349331/LConn1
  T_158349331__/RConn2 -- L_158349331/LConn2
  L_158349331/LConn3 -- T_158349331__/RConn3 -- bus295/LConn1
  T_109525418_220000_Подстанция_220_кВ_Титан/RConn1 -- L_109525418/LConn1
  T_109525418_220000_Подстанция_220_кВ_Титан/RConn2 -- L_109525418/LConn2
  L_109525418/LConn3 -- T_109525418_220000_Подстанция_220_кВ_Титан/RConn3 -- bus296/LConn1
  T_330052123_110000_ПС_110_6_кВ_Прудовая/RConn1 -- L_330052123/LConn1
  T_330052123_110000_ПС_110_6_кВ_Прудовая/RConn2 -- L_330052123/LConn2
  L_330052123/LConn3 -- T_330052123_110000_ПС_110_6_кВ_Прудовая/RConn3 -- bus297/LConn1
  T_116695201_110000_ПС_110_35_6_Воткинск/RConn1 -- L_116695201/LConn1
  T_116695201_110000_ПС_110_35_6_Воткинск/RConn2 -- L_116695201/LConn2
  L_116695201/LConn3 -- T_116695201_110000_ПС_110_35_6_Воткинск/RConn3 -- bus298/LConn1
  T_262366242_110000;35000;10000_ПС_110_35_10_кВ_Батырево/RConn1 -- L_262366242/LConn1
  T_262366242_110000;35000;10000_ПС_110_35_10_кВ_Батырево/RConn2 -- L_262366242/LConn2
  L_262366242/LConn3 -- T_262366242_110000;35000;10000_ПС_110_35_10_кВ_Батырево/RConn3 -- bus299/LConn1
  T_208425687_110000;35000;10000_ПС_110_35_10_кВ_Комсомольская/RConn1 -- L_208425687/LConn1
  T_208425687_110000;35000;10000_ПС_110_35_10_кВ_Комсомольская/RConn2 -- L_208425687/LConn2
  L_208425687/LConn3 -- T_208425687_110000;35000;10000_ПС_110_35_10_кВ_Комсомольская/RConn3 -- bus300/LConn1
  T_243068515_110000;10000_ПС_110_10_кВ_Маяк/RConn1 -- L_243068515/LConn1
  T_243068515_110000;10000_ПС_110_10_кВ_Маяк/RConn2 -- L_243068515/LConn2
  L_243068515/LConn3 -- T_243068515_110000;10000_ПС_110_10_кВ_Маяк/RConn3 -- bus301/LConn1
  T_262366241_110000;10000_ПС_110_10_кВ_Сугуты/RConn1 -- L_262366241/LConn1
  T_262366241_110000;10000_ПС_110_10_кВ_Сугуты/RConn2 -- L_262366241/LConn2
  L_262366241/LConn3 -- T_262366241_110000;10000_ПС_110_10_кВ_Сугуты/RConn3 -- bus302/LConn1
  T_310752804_110000;35000;10000_ПС_«Чапаевская»_110_35_10_кВ/RConn1 -- L_310752804/LConn1
  T_310752804_110000;35000;10000_ПС_«Чапаевская»_110_35_10_кВ/RConn2 -- L_310752804/LConn2
  L_310752804/LConn3 -- T_310752804_110000;35000;10000_ПС_«Чапаевская»_110_35_10_кВ/RConn3 -- bus303/LConn1
  T_243075861_110000;6000_ПС_110_6_кВ_Южная/RConn1 -- L_243075861/LConn1
  T_243075861_110000;6000_ПС_110_6_кВ_Южная/RConn2 -- L_243075861/LConn2
  L_243075861/LConn3 -- T_243075861_110000;6000_ПС_110_6_кВ_Южная/RConn3 -- bus304/LConn1
  T_97124903__/RConn1 -- L_97124903/LConn1
  T_97124903__/RConn2 -- L_97124903/LConn2
  L_97124903/LConn3 -- T_97124903__/RConn3 -- bus305/LConn1
  T_145399632__/RConn1 -- L_145399632/LConn1
  T_145399632__/RConn2 -- L_145399632/LConn2
  L_145399632/LConn3 -- T_145399632__/RConn3 -- bus306/LConn1
  T_97124768__/RConn1 -- L_97124768/LConn1
  T_97124768__/RConn2 -- L_97124768/LConn2
  L_97124768/LConn3 -- T_97124768__/RConn3 -- bus307/LConn1
  T_279978588_110000;10000_ПС_110_10_кВ_Алгаши/RConn1 -- L_279978588/LConn1
  T_279978588_110000;10000_ПС_110_10_кВ_Алгаши/RConn2 -- L_279978588/LConn2
  L_279978588/LConn3 -- T_279978588_110000;10000_ПС_110_10_кВ_Алгаши/RConn3 -- bus308/LConn1
  T_279978582_110000;35000;10000_ПС_110_35_10_кВ_Порецкая/RConn1 -- L_279978582/LConn1
  T_279978582_110000;35000;10000_ПС_110_35_10_кВ_Порецкая/RConn2 -- L_279978582/LConn2
  L_279978582/LConn3 -- T_279978582_110000;35000;10000_ПС_110_35_10_кВ_Порецкая/RConn3 -- bus309/LConn1
  T_279978583_110000;10000_ПС_110_10_кВ_Кожевенная/RConn1 -- L_279978583/LConn1
  T_279978583_110000;10000_ПС_110_10_кВ_Кожевенная/RConn2 -- L_279978583/LConn2
  L_279978583/LConn3 -- T_279978583_110000;10000_ПС_110_10_кВ_Кожевенная/RConn3 -- bus310/LConn1
  T_250911823__ПС_Б_Матаки/RConn1 -- L_250911823/LConn1
  T_250911823__ПС_Б_Матаки/RConn2 -- L_250911823/LConn2
  L_250911823/LConn3 -- T_250911823__ПС_Б_Матаки/RConn3 -- bus311/LConn1
  T_351596015__ПС_Ромодан/RConn1 -- L_351596015/LConn1
  T_351596015__ПС_Ромодан/RConn2 -- L_351596015/LConn2
  L_351596015/LConn3 -- T_351596015__ПС_Ромодан/RConn3 -- bus312/LConn1
  T_183273018__ПС_Салманы/RConn1 -- L_183273018/LConn1
  T_183273018__ПС_Салманы/RConn2 -- L_183273018/LConn2
  L_183273018/LConn3 -- T_183273018__ПС_Салманы/RConn3 -- bus313/LConn1
  T_194431022_110000;35000;10000_ПС_110_35_10_кВ_Яльчики/RConn1 -- L_194431022/LConn1
  T_194431022_110000;35000;10000_ПС_110_35_10_кВ_Яльчики/RConn2 -- L_194431022/LConn2
  L_194431022/LConn3 -- T_194431022_110000;35000;10000_ПС_110_35_10_кВ_Яльчики/RConn3 -- bus314/LConn1
  T_279778884_110000;10000_ПС_110_10_кВ_Слава/RConn1 -- L_279778884/LConn1
  T_279778884_110000;10000_ПС_110_10_кВ_Слава/RConn2 -- L_279778884/LConn2
  L_279778884/LConn3 -- T_279778884_110000;10000_ПС_110_10_кВ_Слава/RConn3 -- bus315/LConn1
  T_172508720_110000_ПС_110_10_Успенка/RConn1 -- L_172508720/LConn1
  T_172508720_110000_ПС_110_10_Успенка/RConn2 -- L_172508720/LConn2
  L_172508720/LConn3 -- T_172508720_110000_ПС_110_10_Успенка/RConn3 -- bus316/LConn1
  T_157080628__/RConn1 -- L_157080628/LConn1
  T_157080628__/RConn2 -- L_157080628/LConn2
  L_157080628/LConn3 -- T_157080628__/RConn3 -- bus317/LConn1
  T_192432407__/RConn1 -- L_192432407/LConn1
  T_192432407__/RConn2 -- L_192432407/LConn2
  L_192432407/LConn3 -- T_192432407__/RConn3 -- bus318/LConn1
  T_192432406__/RConn1 -- L_192432406/LConn1
  T_192432406__/RConn2 -- L_192432406/LConn2
  L_192432406/LConn3 -- T_192432406__/RConn3 -- bus319/LConn1
  T_192426717_110000_ПС_Люзень/RConn1 -- L_192426717/LConn1
  T_192426717_110000_ПС_Люзень/RConn2 -- L_192426717/LConn2
  L_192426717/LConn3 -- T_192426717_110000_ПС_Люзень/RConn3 -- bus320/LConn1
  T_236703070__ПС_Дубъязы/RConn1 -- L_236703070/LConn1
  T_236703070__ПС_Дубъязы/RConn2 -- L_236703070/LConn2
  L_236703070/LConn3 -- T_236703070__ПС_Дубъязы/RConn3 -- bus321/LConn1
  T_180786877__ПС_Алат/RConn1 -- L_180786877/LConn1
  T_180786877__ПС_Алат/RConn2 -- L_180786877/LConn2
  L_180786877/LConn3 -- T_180786877__ПС_Алат/RConn3 -- bus322/LConn1
  T_291372086_110000_пс_Села_110_10кВ/RConn1 -- L_291372086/LConn1
  T_291372086_110000_пс_Села_110_10кВ/RConn2 -- L_291372086/LConn2
  L_291372086/LConn3 -- T_291372086_110000_пс_Села_110_10кВ/RConn3 -- bus323/LConn1
  T_291372085_110000_пс_Кутамыш/RConn1 -- L_291372085/LConn1
  T_291372085_110000_пс_Кутамыш/RConn2 -- L_291372085/LConn2
  L_291372085/LConn3 -- T_291372085_110000_пс_Кутамыш/RConn3 -- bus324/LConn1
  T_277905349_110000;10000_Андреевка/RConn1 -- L_277905349/LConn1
  T_277905349_110000;10000_Андреевка/RConn2 -- L_277905349/LConn2
  L_277905349/LConn3 -- T_277905349_110000;10000_Андреевка/RConn3 -- bus325/LConn1
  T_242972920_110000;10000_ПС_110_10_кВ_Заволжская/RConn1 -- L_242972920/LConn1
  T_242972920_110000;10000_ПС_110_10_кВ_Заволжская/RConn2 -- L_242972920/LConn2
  L_242972920/LConn3 -- T_242972920_110000;10000_ПС_110_10_кВ_Заволжская/RConn3 -- bus326/LConn1
  T_242973735_110000;10000_ПС_110_10_кВ_Яндоба/RConn1 -- L_242973735/LConn1
  T_242973735_110000;10000_ПС_110_10_кВ_Яндоба/RConn2 -- L_242973735/LConn2
  L_242973735/LConn3 -- T_242973735_110000;10000_ПС_110_10_кВ_Яндоба/RConn3 -- bus327/LConn1
  T_292328535_110000;10000_ПС_110_10_кВ_Виловатово/RConn1 -- L_292328535/LConn1
  T_292328535_110000;10000_ПС_110_10_кВ_Виловатово/RConn2 -- L_292328535/LConn2
  L_292328535/LConn3 -- T_292328535_110000;10000_ПС_110_10_кВ_Виловатово/RConn3 -- bus328/LConn1
  T_292068563_110000;35000;10000_ПС_110_35_10_кВ_Еласы/RConn1 -- L_292068563/LConn1
  T_292068563_110000;35000;10000_ПС_110_35_10_кВ_Еласы/RConn2 -- L_292068563/LConn2
  L_292068563/LConn3 -- T_292068563_110000;35000;10000_ПС_110_35_10_кВ_Еласы/RConn3 -- bus329/LConn1
  T_280247964_110000;10000_ПС_110_10_кВ_Сундырь/RConn1 -- L_280247964/LConn1
  T_280247964_110000;10000_ПС_110_10_кВ_Сундырь/RConn2 -- L_280247964/LConn2
  L_280247964/LConn3 -- T_280247964_110000;10000_ПС_110_10_кВ_Сундырь/RConn3 -- bus330/LConn1
  T_226055229_110000;10000_ПС_110_10_кВ_Козловка/RConn1 -- L_226055229/LConn1
  T_226055229_110000;10000_ПС_110_10_кВ_Козловка/RConn2 -- L_226055229/LConn2
  L_226055229/LConn3 -- T_226055229_110000;10000_ПС_110_10_кВ_Козловка/RConn3 -- bus331/LConn1
  T_115651649_110000;10000_ПС_110_10_кВ_Вурманкасы/RConn1 -- L_115651649/LConn1
  T_115651649_110000;10000_ПС_110_10_кВ_Вурманкасы/RConn2 -- L_115651649/LConn2
  L_115651649/LConn3 -- T_115651649_110000;10000_ПС_110_10_кВ_Вурманкасы/RConn3 -- bus332/LConn1
  T_281879368_110000;10000_ПС_110_10_кВ_Радуга/RConn1 -- L_281879368/LConn1
  T_281879368_110000;10000_ПС_110_10_кВ_Радуга/RConn2 -- L_281879368/LConn2
  L_281879368/LConn3 -- T_281879368_110000;10000_ПС_110_10_кВ_Радуга/RConn3 -- bus333/LConn1
  T_281834847_110000;35000;10000_ПС_110_35_10_кВ_Кугеси/RConn1 -- L_281834847/LConn1
  T_281834847_110000;35000;10000_ПС_110_35_10_кВ_Кугеси/RConn2 -- L_281834847/LConn2
  L_281834847/LConn3 -- T_281834847_110000;35000;10000_ПС_110_35_10_кВ_Кугеси/RConn3 -- bus334/LConn1
  T_120823877__ПС_Федоровская/RConn1 -- L_120823877/LConn1
  T_120823877__ПС_Федоровская/RConn2 -- L_120823877/LConn2
  L_120823877/LConn3 -- T_120823877__ПС_Федоровская/RConn3 -- bus335/LConn1
  T_229841888__ПС_Нурлаты/RConn1 -- L_229841888/LConn1
  T_229841888__ПС_Нурлаты/RConn2 -- L_229841888/LConn2
  L_229841888/LConn3 -- T_229841888__ПС_Нурлаты/RConn3 -- bus336/LConn1
  T_171977680__ПС_Апастово/RConn1 -- L_171977680/LConn1
  T_171977680__ПС_Апастово/RConn2 -- L_171977680/LConn2
  L_171977680/LConn3 -- T_171977680__ПС_Апастово/RConn3 -- bus337/LConn1
  T_176838936__ПС_Каратун/RConn1 -- L_176838936/LConn1
  T_176838936__ПС_Каратун/RConn2 -- L_176838936/LConn2
  L_176838936/LConn3 -- T_176838936__ПС_Каратун/RConn3 -- bus338/LConn1
  T_94242892__Подстанция_№3/RConn1 -- L_94242892/LConn1
  T_94242892__Подстанция_№3/RConn2 -- L_94242892/LConn2
  L_94242892/LConn3 -- T_94242892__Подстанция_№3/RConn3 -- bus339/LConn1
  "T_138632781_220000;110000;10000_ПС_220_110_10_кВ_\"Сасово\""/RConn1 -- L_138632781/LConn1
  "T_138632781_220000;110000;10000_ПС_220_110_10_кВ_\"Сасово\""/RConn2 -- L_138632781/LConn2
  L_138632781/LConn3 -- "T_138632781_220000;110000;10000_ПС_220_110_10_кВ_\"Сасово\""/RConn3 -- bus340/LConn1
  "T_138722426__ПС_110_10кВ_\"Вад\""/RConn1 -- L_138722426/LConn1
  "T_138722426__ПС_110_10кВ_\"Вад\""/RConn2 -- L_138722426/LConn2
  L_138722426/LConn3 -- "T_138722426__ПС_110_10кВ_\"Вад\""/RConn3 -- bus341/LConn1
  T_140944227__/RConn1 -- L_140944227/LConn1
  T_140944227__/RConn2 -- L_140944227/LConn2
  L_140944227/LConn3 -- T_140944227__/RConn3 -- bus342/LConn1
  "T_140940409_110000;10000_ПС_110_10_кВ_\"Свобода\""/RConn1 -- L_140940409/LConn1
  "T_140940409_110000;10000_ПС_110_10_кВ_\"Свобода\""/RConn2 -- L_140940409/LConn2
  L_140940409/LConn3 -- "T_140940409_110000;10000_ПС_110_10_кВ_\"Свобода\""/RConn3 -- bus343/LConn1
  "T_181334375__ПС_110_10кВ_\"Кустаревка\""/RConn1 -- L_181334375/LConn1
  "T_181334375__ПС_110_10кВ_\"Кустаревка\""/RConn2 -- L_181334375/LConn2
  L_181334375/LConn3 -- "T_181334375__ПС_110_10кВ_\"Кустаревка\""/RConn3 -- bus344/LConn1
  T_313773134_110000;35000;6000_ПС_110_35_6_кВ_Порт/RConn1 -- L_313773134/LConn1
  T_313773134_110000;35000;6000_ПС_110_35_6_кВ_Порт/RConn2 -- L_313773134/LConn2
  L_313773134/LConn3 -- T_313773134_110000;35000;6000_ПС_110_35_6_кВ_Порт/RConn3 -- bus345/LConn1
  T_313773131__/RConn1 -- L_313773131/LConn1
  T_313773131__/RConn2 -- L_313773131/LConn2
  L_313773131/LConn3 -- T_313773131__/RConn3 -- bus346/LConn1
  T_226054226_110000;10000_ПС_110_10_кВ_Кибечи/RConn1 -- L_226054226/LConn1
  T_226054226_110000;10000_ПС_110_10_кВ_Кибечи/RConn2 -- L_226054226/LConn2
  L_226054226/LConn3 -- T_226054226_110000;10000_ПС_110_10_кВ_Кибечи/RConn3 -- bus347/LConn1
  T_226052064_110000;10000_ПС_110_10_кВ_Шоркистры/RConn1 -- L_226052064/LConn1
  T_226052064_110000;10000_ПС_110_10_кВ_Шоркистры/RConn2 -- L_226052064/LConn2
  L_226052064/LConn3 -- T_226052064_110000;10000_ПС_110_10_кВ_Шоркистры/RConn3 -- bus348/LConn1
  T_243069892_110000;35000;10000_ПС_110_35_10_кВ_Урмары/RConn1 -- L_243069892/LConn1
  T_243069892_110000;35000;10000_ПС_110_35_10_кВ_Урмары/RConn2 -- L_243069892/LConn2
  L_243069892/LConn3 -- T_243069892_110000;35000;10000_ПС_110_35_10_кВ_Урмары/RConn3 -- bus349/LConn1
  T_279978581_110000;10000_ПС_110_10_кВ_Кувакино/RConn1 -- L_279978581/LConn1
  T_279978581_110000;10000_ПС_110_10_кВ_Кувакино/RConn2 -- L_279978581/LConn2
  L_279978581/LConn3 -- T_279978581_110000;10000_ПС_110_10_кВ_Кувакино/RConn3 -- bus350/LConn1
  T_222133214_110000;10000_ПС_110_10_кВ_Семеновская/RConn1 -- L_222133214/LConn1
  T_222133214_110000;10000_ПС_110_10_кВ_Семеновская/RConn2 -- L_222133214/LConn2
  L_222133214/LConn3 -- T_222133214_110000;10000_ПС_110_10_кВ_Семеновская/RConn3 -- bus351/LConn1
  T_108403292__/RConn1 -- L_108403292/LConn1
  T_108403292__/RConn2 -- L_108403292/LConn2
  L_108403292/LConn3 -- T_108403292__/RConn3 -- bus352/LConn1
  T_193928464__ПС_КПД/RConn1 -- L_193928464/LConn1
  T_193928464__ПС_КПД/RConn2 -- L_193928464/LConn2
  L_193928464/LConn3 -- T_193928464__ПС_КПД/RConn3 -- bus353/LConn1
  T_102447718__/RConn1 -- L_102447718/LConn1
  T_102447718__/RConn2 -- L_102447718/LConn2
  L_102447718/LConn3 -- T_102447718__/RConn3 -- bus354/LConn1
  T_308883878__/RConn1 -- L_308883878/LConn1
  T_308883878__/RConn2 -- L_308883878/LConn2
  L_308883878/LConn3 -- T_308883878__/RConn3 -- bus355/LConn1
  T_279258960_110000;35000;10000_ПС_110_35_10_кВ_Красноармейская/RConn1 -- L_279258960/LConn1
  T_279258960_110000;35000;10000_ПС_110_35_10_кВ_Красноармейская/RConn2 -- L_279258960/LConn2
  L_279258960/LConn3 -- T_279258960_110000;35000;10000_ПС_110_35_10_кВ_Красноармейская/RConn3 -- bus356/LConn1
  T_241262030_110000;35000;10000_ПС_110_35_10_кВ_Цивильск/RConn1 -- L_241262030/LConn1
  T_241262030_110000;35000;10000_ПС_110_35_10_кВ_Цивильск/RConn2 -- L_241262030/LConn2
  L_241262030/LConn3 -- T_241262030_110000;35000;10000_ПС_110_35_10_кВ_Цивильск/RConn3 -- bus357/LConn1
  T_242932802_110000;10000_ПС_110_10_кВ_Оросительная/RConn1 -- L_242932802/LConn1
  T_242932802_110000;10000_ПС_110_10_кВ_Оросительная/RConn2 -- L_242932802/LConn2
  L_242932802/LConn3 -- T_242932802_110000;10000_ПС_110_10_кВ_Оросительная/RConn3 -- bus358/LConn1
  T_110255218__ПС_Кожино_110_35кВ/RConn1 -- L_110255218/LConn1
  T_110255218__ПС_Кожино_110_35кВ/RConn2 -- L_110255218/LConn2
  L_110255218/LConn3 -- T_110255218__ПС_Кожино_110_35кВ/RConn3 -- bus359/LConn1
  T_330006647_110000_/RConn1 -- L_330006647/LConn1
  T_330006647_110000_/RConn2 -- L_330006647/LConn2
  L_330006647/LConn3 -- T_330006647_110000_/RConn3 -- bus360/LConn1
  T_57948286_110000;10000_Сазанлей/RConn1 -- L_57948286/LConn1
  T_57948286_110000;10000_Сазанлей/RConn2 -- L_57948286/LConn2
  L_57948286/LConn3 -- T_57948286_110000;10000_Сазанлей/RConn3 -- bus361/LConn1
  T_51711248_110000_/RConn1 -- L_51711248/LConn1
  T_51711248_110000_/RConn2 -- L_51711248/LConn2
  L_51711248/LConn3 -- T_51711248_110000_/RConn3 -- bus362/LConn1
  "T_51601242_220000;110000;fixme_ПС_220_кВ_\"Центральная\""/RConn1 -- L_51601242/LConn1
  "T_51601242_220000;110000;fixme_ПС_220_кВ_\"Центральная\""/RConn2 -- L_51601242/LConn2
  L_51601242/LConn3 -- "T_51601242_220000;110000;fixme_ПС_220_кВ_\"Центральная\""/RConn3 -- bus363/LConn1
  T_244847744__/RConn1 -- L_244847744/LConn1
  T_244847744__/RConn2 -- L_244847744/LConn2
  L_244847744/LConn3 -- T_244847744__/RConn3 -- bus364/LConn1
  T_279846258_110000;10000_ПС_110_10_кВ_Ачаксы/RConn1 -- L_279846258/LConn1
  T_279846258_110000;10000_ПС_110_10_кВ_Ачаксы/RConn2 -- L_279846258/LConn2
  L_279846258/LConn3 -- T_279846258_110000;10000_ПС_110_10_кВ_Ачаксы/RConn3 -- bus365/LConn1
  T_280247940_110000;10000_ПС_110_10_кВ_Саланчики/RConn1 -- L_280247940/LConn1
  T_280247940_110000;10000_ПС_110_10_кВ_Саланчики/RConn2 -- L_280247940/LConn2
  L_280247940/LConn3 -- T_280247940_110000;10000_ПС_110_10_кВ_Саланчики/RConn3 -- bus366/LConn1
  T_280247942_110000;35000;10000_ПС_110_35_10_кВ_Красночетайская/RConn1 -- L_280247942/LConn1
  T_280247942_110000;35000;10000_ПС_110_35_10_кВ_Красночетайская/RConn2 -- L_280247942/LConn2
  L_280247942/LConn3 -- T_280247942_110000;35000;10000_ПС_110_35_10_кВ_Красночетайская/RConn3 -- bus367/LConn1
  T_280247938__/RConn1 -- L_280247938/LConn1
  T_280247938__/RConn2 -- L_280247938/LConn2
  L_280247938/LConn3 -- T_280247938__/RConn3 -- bus368/LConn1
  T_207206840__Тяговая_подстанция/RConn1 -- L_207206840/LConn1
  T_207206840__Тяговая_подстанция/RConn2 -- L_207206840/LConn2
  L_207206840/LConn3 -- T_207206840__Тяговая_подстанция/RConn3 -- bus369/LConn1
  "T_56048772_220000_Электрическая_подстанция_\"Горная\""/RConn1 -- L_56048772/LConn1
  "T_56048772_220000_Электрическая_подстанция_\"Горная\""/RConn2 -- L_56048772/LConn2
  L_56048772/LConn3 -- "T_56048772_220000_Электрическая_подстанция_\"Горная\""/RConn3 -- bus370/LConn1
  T_53566695__Подстанция_Кизел_(ж_д)/RConn1 -- L_53566695/LConn1
  T_53566695__Подстанция_Кизел_(ж_д)/RConn2 -- L_53566695/LConn2
  L_53566695/LConn3 -- T_53566695__Подстанция_Кизел_(ж_д)/RConn3 -- bus371/LConn1
  T_116695174_110000_ПС_110_6_кВ_Инструментальная/RConn1 -- L_116695174/LConn1
  T_116695174_110000_ПС_110_6_кВ_Инструментальная/RConn2 -- L_116695174/LConn2
  L_116695174/LConn3 -- T_116695174_110000_ПС_110_6_кВ_Инструментальная/RConn3 -- bus372/LConn1
  T_191841753__ПС_Свияжск/RConn1 -- L_191841753/LConn1
  T_191841753__ПС_Свияжск/RConn2 -- L_191841753/LConn2
  L_191841753/LConn3 -- T_191841753__ПС_Свияжск/RConn3 -- bus373/LConn1
  T_226055643__/RConn1 -- L_226055643/LConn1
  T_226055643__/RConn2 -- L_226055643/LConn2
  L_226055643/LConn3 -- T_226055643__/RConn3 -- bus374/LConn1
  T_280247955_110000;35000;10000_ПС_110_35_10_кВ_Кукшум/RConn1 -- L_280247955/LConn1
  T_280247955_110000;35000;10000_ПС_110_35_10_кВ_Кукшум/RConn2 -- L_280247955/LConn2
  L_280247955/LConn3 -- T_280247955_110000;35000;10000_ПС_110_35_10_кВ_Кукшум/RConn3 -- bus375/LConn1
  T_280247957_110000;35000;10000_ПС_110_35_10_кВ_ЯМЗ/RConn1 -- L_280247957/LConn1
  T_280247957_110000;35000;10000_ПС_110_35_10_кВ_ЯМЗ/RConn2 -- L_280247957/LConn2
  L_280247957/LConn3 -- T_280247957_110000;35000;10000_ПС_110_35_10_кВ_ЯМЗ/RConn3 -- bus376/LConn1
  T_315675920_110000;10000_ПС_Покров_Майдан_110_10_кВ/RConn1 -- L_315675920/LConn1
  T_315675920_110000;10000_ПС_Покров_Майдан_110_10_кВ/RConn2 -- L_315675920/LConn2
  L_315675920/LConn3 -- T_315675920_110000;10000_ПС_Покров_Майдан_110_10_кВ/RConn3 -- bus377/LConn1
  T_107943661_110000_Медведевский_электроучасток/RConn1 -- L_107943661/LConn1
  T_107943661_110000_Медведевский_электроучасток/RConn2 -- L_107943661/LConn2
  L_107943661/LConn3 -- T_107943661_110000_Медведевский_электроучасток/RConn3 -- bus378/LConn1
  T_176859804__Жасминная/RConn1 -- L_176859804/LConn1
  T_176859804__Жасминная/RConn2 -- L_176859804/LConn2
  L_176859804/LConn3 -- T_176859804__Жасминная/RConn3 -- bus379/LConn1
  T_176642248__Елшанка_2/RConn1 -- L_176642248/LConn1
  T_176642248__Елшанка_2/RConn2 -- L_176642248/LConn2
  L_176642248/LConn3 -- T_176642248__Елшанка_2/RConn3 -- bus380/LConn1
  T_243531233__ПС_Малмыж/RConn1 -- L_243531233/LConn1
  T_243531233__ПС_Малмыж/RConn2 -- L_243531233/LConn2
  L_243531233/LConn3 -- T_243531233__ПС_Малмыж/RConn3 -- bus381/LConn1
  T_247403714__ПС_Сардек/RConn1 -- L_247403714/LConn1
  T_247403714__ПС_Сардек/RConn2 -- L_247403714/LConn2
  L_247403714/LConn3 -- T_247403714__ПС_Сардек/RConn3 -- bus382/LConn1
  T_110370987__ПС_Краснооктябрьск_110_10кВ/RConn1 -- L_110370987/LConn1
  T_110370987__ПС_Краснооктябрьск_110_10кВ/RConn2 -- L_110370987/LConn2
  L_110370987/LConn3 -- T_110370987__ПС_Краснооктябрьск_110_10кВ/RConn3 -- bus383/LConn1
  T_112681450_110000_/RConn1 -- L_112681450/LConn1
  T_112681450_110000_/RConn2 -- L_112681450/LConn2
  L_112681450/LConn3 -- T_112681450_110000_/RConn3 -- bus384/LConn1
  T_319459210__/RConn1 -- L_319459210/LConn1
  T_319459210__/RConn2 -- L_319459210/LConn2
  L_319459210/LConn3 -- T_319459210__/RConn3 -- bus385/LConn1
  T_319459220_110000;10000_Перемская/RConn1 -- L_319459220/LConn1
  T_319459220_110000;10000_Перемская/RConn2 -- L_319459220/LConn2
  L_319459220/LConn3 -- T_319459220_110000;10000_Перемская/RConn3 -- bus386/LConn1
  T_243154612__/RConn1 -- L_243154612/LConn1
  T_243154612__/RConn2 -- L_243154612/LConn2
  L_243154612/LConn3 -- T_243154612__/RConn3 -- bus387/LConn1
  T_243820930__/RConn1 -- L_243820930/LConn1
  T_243820930__/RConn2 -- L_243820930/LConn2
  L_243820930/LConn3 -- T_243820930__/RConn3 -- bus388/LConn1
  T_97060032__/RConn1 -- L_97060032/LConn1
  T_97060032__/RConn2 -- L_97060032/LConn2
  L_97060032/LConn3 -- T_97060032__/RConn3 -- bus389/LConn1
  T_97060037__/RConn1 -- L_97060037/LConn1
  T_97060037__/RConn2 -- L_97060037/LConn2
  L_97060037/LConn3 -- T_97060037__/RConn3 -- bus390/LConn1
  T_100584516__/RConn1 -- L_100584516/LConn1
  T_100584516__/RConn2 -- L_100584516/LConn2
  L_100584516/LConn3 -- T_100584516__/RConn3 -- bus391/LConn1
  "T_327245366_110000_ПС_110_10кВ_\"Разино\""/RConn1 -- L_327245366/LConn1
  "T_327245366_110000_ПС_110_10кВ_\"Разино\""/RConn2 -- L_327245366/LConn2
  L_327245366/LConn3 -- "T_327245366_110000_ПС_110_10кВ_\"Разино\""/RConn3 -- bus392/LConn1
  "T_305832833_110000_ПС_110_10кВ_\"Мадаево\""/RConn1 -- L_305832833/LConn1
  "T_305832833_110000_ПС_110_10кВ_\"Мадаево\""/RConn2 -- L_305832833/LConn2
  L_305832833/LConn3 -- "T_305832833_110000_ПС_110_10кВ_\"Мадаево\""/RConn3 -- bus393/LConn1
  T_106289362__/RConn1 -- L_106289362/LConn1
  T_106289362__/RConn2 -- L_106289362/LConn2
  L_106289362/LConn3 -- T_106289362__/RConn3 -- bus394/LConn1
  T_106289442__/RConn1 -- L_106289442/LConn1
  T_106289442__/RConn2 -- L_106289442/LConn2
  L_106289442/LConn3 -- T_106289442__/RConn3 -- bus395/LConn1
  T_55334100__/RConn1 -- L_55334100/LConn1
  T_55334100__/RConn2 -- L_55334100/LConn2
  L_55334100/LConn3 -- T_55334100__/RConn3 -- bus396/LConn1
  T_55334115__/RConn1 -- L_55334115/LConn1
  T_55334115__/RConn2 -- L_55334115/LConn2
  L_55334115/LConn3 -- T_55334115__/RConn3 -- bus397/LConn1
  "T_327245584_110000_ПС_110_10кВ_\"Лукоянов_110\""/RConn1 -- L_327245584/LConn1
  "T_327245584_110000_ПС_110_10кВ_\"Лукоянов_110\""/RConn2 -- L_327245584/LConn2
  L_327245584/LConn3 -- "T_327245584_110000_ПС_110_10кВ_\"Лукоянов_110\""/RConn3 -- bus398/LConn1
  "T_327245371_110000_ПС_110_35_10кВ_\"Починки_110\""/RConn1 -- L_327245371/LConn1
  "T_327245371_110000_ПС_110_35_10кВ_\"Починки_110\""/RConn2 -- L_327245371/LConn2
  L_327245371/LConn3 -- "T_327245371_110000_ПС_110_35_10кВ_\"Починки_110\""/RConn3 -- bus399/LConn1
  T_58880346_110000;35000;10000_ПС_110_35_10_кВ_Спутник/RConn1 -- L_58880346/LConn1
  T_58880346_110000;35000;10000_ПС_110_35_10_кВ_Спутник/RConn2 -- L_58880346/LConn2
  L_58880346/LConn3 -- T_58880346_110000;35000;10000_ПС_110_35_10_кВ_Спутник/RConn3 -- bus400/LConn1
  T_281879365_110000;10000_ПС_110_10_кВ_Светлая/RConn1 -- L_281879365/LConn1
  T_281879365_110000;10000_ПС_110_10_кВ_Светлая/RConn2 -- L_281879365/LConn2
  L_281879365/LConn3 -- T_281879365_110000;10000_ПС_110_10_кВ_Светлая/RConn3 -- bus401/LConn1
  T_337947383__/RConn1 -- L_337947383/LConn1
  T_337947383__/RConn2 -- L_337947383/LConn2
  L_337947383/LConn3 -- T_337947383__/RConn3 -- bus402/LConn1
  T_90868997__/RConn1 -- L_90868997/LConn1
  T_90868997__/RConn2 -- L_90868997/LConn2
  L_90868997/LConn3 -- T_90868997__/RConn3 -- bus403/LConn1
  T_211578632_110000_ПС_СИЛЬВИНИТ/RConn1 -- L_211578632/LConn1
  T_211578632_110000_ПС_СИЛЬВИНИТ/RConn2 -- L_211578632/LConn2
  L_211578632/LConn3 -- T_211578632_110000_ПС_СИЛЬВИНИТ/RConn3 -- bus404/LConn1
  T_307428692__Сибирь/RConn1 -- L_307428692/LConn1
  T_307428692__Сибирь/RConn2 -- L_307428692/LConn2
  L_307428692/LConn3 -- T_307428692__Сибирь/RConn3 -- bus405/LConn1
  T_245404985_110000_ПС_Уньва/RConn1 -- L_245404985/LConn1
  T_245404985_110000_ПС_Уньва/RConn2 -- L_245404985/LConn2
  L_245404985/LConn3 -- T_245404985_110000_ПС_Уньва/RConn3 -- bus406/LConn1
  T_286921936__/RConn1 -- L_286921936/LConn1
  T_286921936__/RConn2 -- L_286921936/LConn2
  L_286921936/LConn3 -- T_286921936__/RConn3 -- bus407/LConn1
  T_109525394_220000_ПС_220_кВ_Калийная/RConn1 -- L_109525394/LConn1
  T_109525394_220000_ПС_220_кВ_Калийная/RConn2 -- L_109525394/LConn2
  L_109525394/LConn3 -- T_109525394_220000_ПС_220_кВ_Калийная/RConn3 -- bus408/LConn1
  T_103877395__/RConn1 -- L_103877395/LConn1
  T_103877395__/RConn2 -- L_103877395/LConn2
  L_103877395/LConn3 -- T_103877395__/RConn3 -- bus409/LConn1
  T_103877470__/RConn1 -- L_103877470/LConn1
  T_103877470__/RConn2 -- L_103877470/LConn2
  L_103877470/LConn3 -- T_103877470__/RConn3 -- bus410/LConn1
  T_287462706_110000_110_КВ_Тёплая_Гора/RConn1 -- L_287462706/LConn1
  T_287462706_110000_110_КВ_Тёплая_Гора/RConn2 -- L_287462706/LConn2
  L_287462706/LConn3 -- T_287462706_110000_110_КВ_Тёплая_Гора/RConn3 -- bus411/LConn1
  T_238317576__/RConn1 -- L_238317576/LConn1
  T_238317576__/RConn2 -- L_238317576/LConn2
  L_238317576/LConn3 -- T_238317576__/RConn3 -- bus412/LConn1
  T_252815158_110000;35000;10000_/RConn1 -- L_252815158/LConn1
  T_252815158_110000;35000;10000_/RConn2 -- L_252815158/LConn2
  L_252815158/LConn3 -- T_252815158_110000;35000;10000_/RConn3 -- bus413/LConn1
  T_252815157__/RConn1 -- L_252815157/LConn1
  T_252815157__/RConn2 -- L_252815157/LConn2
  L_252815157/LConn3 -- T_252815157__/RConn3 -- bus414/LConn1
  T_290776375_110000_ПС_ЗАГОТОВКА/RConn1 -- L_290776375/LConn1
  T_290776375_110000_ПС_ЗАГОТОВКА/RConn2 -- L_290776375/LConn2
  L_290776375/LConn3 -- T_290776375_110000_ПС_ЗАГОТОВКА/RConn3 -- bus415/LConn1
  T_290777752_110000_ГРЕМЯЧАЯ_I/RConn1 -- L_290777752/LConn1
  T_290777752_110000_ГРЕМЯЧАЯ_I/RConn2 -- L_290777752/LConn2
  L_290777752/LConn3 -- T_290777752_110000_ГРЕМЯЧАЯ_I/RConn3 -- bus416/LConn1
  T_93482493__/RConn1 -- L_93482493/LConn1
  T_93482493__/RConn2 -- L_93482493/LConn2
  L_93482493/LConn3 -- T_93482493__/RConn3 -- bus417/LConn1
  T_242610017_110000;35000;10000_ПС_110_35_10_кВ_Лесная/RConn1 -- L_242610017/LConn1
  T_242610017_110000;35000;10000_ПС_110_35_10_кВ_Лесная/RConn2 -- L_242610017/LConn2
  L_242610017/LConn3 -- T_242610017_110000;35000;10000_ПС_110_35_10_кВ_Лесная/RConn3 -- bus418/LConn1
  T_242614771_110000;6000_ПС_110_6_кВ_Тормозная/RConn1 -- L_242614771/LConn1
  T_242614771_110000;6000_ПС_110_6_кВ_Тормозная/RConn2 -- L_242614771/LConn2
  L_242614771/LConn3 -- T_242614771_110000;6000_ПС_110_6_кВ_Тормозная/RConn3 -- bus419/LConn1
  T_207740804_110000;10000_ПС_110_10_кВ_Дружба/RConn1 -- L_207740804/LConn1
  T_207740804_110000;10000_ПС_110_10_кВ_Дружба/RConn2 -- L_207740804/LConn2
  L_207740804/LConn3 -- T_207740804_110000;10000_ПС_110_10_кВ_Дружба/RConn3 -- bus420/LConn1
  T_279846262_110000;10000_ПС_110_10_кВ_Атнашево/RConn1 -- L_279846262/LConn1
  T_279846262_110000;10000_ПС_110_10_кВ_Атнашево/RConn2 -- L_279846262/LConn2
  L_279846262/LConn3 -- T_279846262_110000;10000_ПС_110_10_кВ_Атнашево/RConn3 -- bus421/LConn1
  T_113994637__ПС_Буинск/RConn1 -- L_113994637/LConn1
  T_113994637__ПС_Буинск/RConn2 -- L_113994637/LConn2
  L_113994637/LConn3 -- T_113994637__ПС_Буинск/RConn3 -- bus422/LConn1
  T_109525439__/RConn1 -- L_109525439/LConn1
  T_109525439__/RConn2 -- L_109525439/LConn2
  L_109525439/LConn3 -- T_109525439__/RConn3 -- bus423/LConn1
  T_109525404__/RConn1 -- L_109525404/LConn1
  T_109525404__/RConn2 -- L_109525404/LConn2
  L_109525404/LConn3 -- T_109525404__/RConn3 -- bus424/LConn1
  T_172819864__Содовая_1_110_35_6/RConn1 -- L_172819864/LConn1
  T_172819864__Содовая_1_110_35_6/RConn2 -- L_172819864/LConn2
  L_172819864/LConn3 -- T_172819864__Содовая_1_110_35_6/RConn3 -- bus425/LConn1
  T_190492574__/RConn1 -- L_190492574/LConn1
  T_190492574__/RConn2 -- L_190492574/LConn2
  L_190492574/LConn3 -- T_190492574__/RConn3 -- bus426/LConn1
  T_108913072_110000;10000_Подстанция/RConn1 -- L_108913072/LConn1
  T_108913072_110000;10000_Подстанция/RConn2 -- L_108913072/LConn2
  L_108913072/LConn3 -- T_108913072_110000;10000_Подстанция/RConn3 -- bus427/LConn1
  T_70186926_110000;fixme_Дубравная/RConn1 -- L_70186926/LConn1
  T_70186926_110000;fixme_Дубравная/RConn2 -- L_70186926/LConn2
  L_70186926/LConn3 -- T_70186926_110000;fixme_Дубравная/RConn3 -- bus428/LConn1
  T_70186927_110000;fixme_ЗКПД/RConn1 -- L_70186927/LConn1
  T_70186927_110000;fixme_ЗКПД/RConn2 -- L_70186927/LConn2
  L_70186927/LConn3 -- T_70186927_110000;fixme_ЗКПД/RConn3 -- bus429/LConn1
  T_136761822_110000_/RConn1 -- L_136761822/LConn1
  T_136761822_110000_/RConn2 -- L_136761822/LConn2
  L_136761822/LConn3 -- T_136761822_110000_/RConn3 -- bus430/LConn1
  T_274998912_220000_Мокша/RConn1 -- L_274998912/LConn1
  T_274998912_220000_Мокша/RConn2 -- L_274998912/LConn2
  L_274998912/LConn3 -- T_274998912_220000_Мокша/RConn3 -- bus431/LConn1
  T_113585698_220000_ПС_220кВ_Рузаевка/RConn1 -- L_113585698/LConn1
  T_113585698_220000_ПС_220кВ_Рузаевка/RConn2 -- L_113585698/LConn2
  L_113585698/LConn3 -- T_113585698_220000_ПС_220кВ_Рузаевка/RConn3 -- bus432/LConn1
  T_327816066_220000_Кузнецк/RConn1 -- L_327816066/LConn1
  T_327816066_220000_Кузнецк/RConn2 -- L_327816066/LConn2
  L_327816066/LConn3 -- T_327816066_220000_Кузнецк/RConn3 -- bus433/LConn1
  T_211405161_220000_Пенза_1/RConn1 -- L_211405161/LConn1
  T_211405161_220000_Пенза_1/RConn2 -- L_211405161/LConn2
  L_211405161/LConn3 -- T_211405161_220000_Пенза_1/RConn3 -- bus434/LConn1
  T_305893253_220000;10000_ПС_Абашево_220_10_кВ/RConn1 -- L_305893253/LConn1
  T_305893253_220000;10000_ПС_Абашево_220_10_кВ/RConn2 -- L_305893253/LConn2
  L_305893253/LConn3 -- T_305893253_220000;10000_ПС_Абашево_220_10_кВ/RConn3 -- bus435/LConn1
  T_305832836_220000_Лукояновская/RConn1 -- L_305832836/LConn1
  T_305832836_220000_Лукояновская/RConn2 -- L_305832836/LConn2
  L_305832836/LConn3 -- T_305832836_220000_Лукояновская/RConn3 -- bus436/LConn1
  T_232164616__/RConn1 -- L_232164616/LConn1
  T_232164616__/RConn2 -- L_232164616/LConn2
  L_232164616/LConn3 -- T_232164616__/RConn3 -- bus437/LConn1
  T_229942593__/RConn1 -- L_229942593/LConn1
  T_229942593__/RConn2 -- L_229942593/LConn2
  L_229942593/LConn3 -- T_229942593__/RConn3 -- bus438/LConn1
  T_274937610_220000_ПС_220_кВ_Головная/RConn1 -- L_274937610/LConn1
  T_274937610_220000_ПС_220_кВ_Головная/RConn2 -- L_274937610/LConn2
  L_274937610/LConn3 -- T_274937610_220000_ПС_220_кВ_Головная/RConn3 -- bus439/LConn1
  T_93494543_220000_Сеченово_1/RConn1 -- L_93494543/LConn1
  T_93494543_220000_Сеченово_1/RConn2 -- L_93494543/LConn2
  L_93494543/LConn3 -- T_93494543_220000_Сеченово_1/RConn3 -- bus440/LConn1
  T_93508340_220000_Сеченово_2/RConn1 -- L_93508340/LConn1
  T_93508340_220000_Сеченово_2/RConn2 -- L_93508340/LConn2
  L_93508340/LConn3 -- T_93508340_220000_Сеченово_2/RConn3 -- bus441/LConn1
  T_93494546_220000_РП_Сеченово/RConn1 -- L_93494546/LConn1
  T_93494546_220000_РП_Сеченово/RConn2 -- L_93494546/LConn2
  L_93494546/LConn3 -- T_93494546_220000_РП_Сеченово/RConn3 -- bus442/LConn1
  T_62194541_220000_ПС_Магистральная/RConn1 -- L_62194541/LConn1
  T_62194541_220000_ПС_Магистральная/RConn2 -- L_62194541/LConn2
  L_62194541/LConn3 -- T_62194541_220000_ПС_Магистральная/RConn3 -- bus443/LConn1
  "T_327138157_220000_ПС_220кВ_\"Пильна\""/RConn1 -- L_327138157/LConn1
  "T_327138157_220000_ПС_220кВ_\"Пильна\""/RConn2 -- L_327138157/LConn2
  L_327138157/LConn3 -- "T_327138157_220000_ПС_220кВ_\"Пильна\""/RConn3 -- bus444/LConn1
  T_224208787_220000_ПС_Дубники/RConn1 -- L_224208787/LConn1
  T_224208787_220000_ПС_Дубники/RConn2 -- L_224208787/LConn2
  L_224208787/LConn3 -- T_224208787_220000_ПС_Дубники/RConn3 -- bus445/LConn1
  T_327325460_220000_Кудьма/RConn1 -- L_327325460/LConn1
  T_327325460_220000_Кудьма/RConn2 -- L_327325460/LConn2
  L_327325460/LConn3 -- T_327325460_220000_Кудьма/RConn3 -- bus446/LConn1
  "T_121048356_220000_ПС_220кВ_\"Бобыльская\""/RConn1 -- L_121048356/LConn1
  "T_121048356_220000_ПС_220кВ_\"Бобыльская\""/RConn2 -- L_121048356/LConn2
  L_121048356/LConn3 -- "T_121048356_220000_ПС_220кВ_\"Бобыльская\""/RConn3 -- bus447/LConn1
  T_171147802__/RConn1 -- L_171147802/LConn1
  T_171147802__/RConn2 -- L_171147802/LConn2
  L_171147802/LConn3 -- T_171147802__/RConn3 -- bus448/LConn1
